simulink model "MRG1x_17B_ERP_030_00_Star23_xx_M256xx_910_x64_RB_Test"  (Simulink 7.8)
settings: Solver=ode45  SolverMode=SingleTasking  StartTime=0.0  StopTime=10.0  RelTol=1e-3
PreLoadFcn:
  | MRG1x_17B_ERP_030_00_Star23_xx_M256xx_910_x64_InitFcn
undefined symbols (not defined in the file or in its folder): ECM
(part 2 of 2)

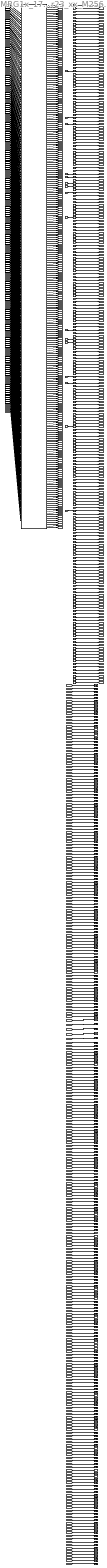
== system MRG1x_17B_ERP_030_00_Star23_xx_M256xx_910_x64_RB_Test/MRG1x_17B_ERP_030_00_Star23_xx_M256xx_910_x64_wrapper ==
  AAP : Inport
  AC_HtrVlv_Front_Req : Inport  Port=2
  AGC_ASSStop_Mode : Inport  Port=3
  AGC_DTREngCutOff_Mode : Inport  Port=4
  AGKInit_Mode : Inport  Port=5
  APP : Inport  Port=6
  AT2_Mode : Inport  Port=7
  AdapAltitudeTempCorr_Coef : Inport  Port=8
  AirFilOutTp_Tp : Inport  Port=9
  AmbAirP_P : Inport  Port=10
  AmbAirTp_Tp : Inport  Port=11
  Bat_Volt : Inport  Port=12
  CacInTp_Tp : Inport  Port=13
  DFI_OprState : Inport  Port=14
  DFSO_Mode : Inport  Port=15
  Dspl_EngShutOff_Time : Inport  Port=16
  ECT : Inport  Port=17
  ECTOut : Inport  Port=18
  ECU_Temp : Inport  Port=19
  EM2_Cool_Req : Inport  Port=20
  EM2_InvrtTemp : Inport  Port=21
  Ecu_St : Inport  Port=22
  Emmo_VoltLinkPN48 : Inport  Port=23
  EngClpmp_FlgOnReq : Inport  Port=24
  EngClpmp_PercPwrReq : Inport  Port=25
  EngCoolTp_Tp : Inport  Port=26
  EngCoolTp_TpMdl : Inport  Port=27
  EngOilP_P : Inport  Port=28
  EngOilTp_Tp : Inport  Port=29
  EngShutOff_Time : Inport  Port=30
  Eng_Actl_OpMode : Inport  Port=31
  Eng_Cyc_Time : Inport  Port=32
  Eng_Fuel_Mass_Flow_Calc : Inport  Port=33
  Eng_RelLoad : Inport  Port=34
  Eng_RelLoad_Req : Inport  Port=35
  Eng_Run_Mode : Inport  Port=36
  Eng_Spd : Inport  Port=37
  Eng_State_Actl : Inport  Port=38
  Eng_Trq : Inport  Port=39
  Eng_Trq_Ind : Inport  Port=40
  Err_ECT_low : Inport  Port=41
  Exh_Temp : Inport  Port=42
  ExtAir_Temp_Raw : Inport  Port=43
  FRT_Sens : Inport  Port=44
  FirstStrt_Mode_EE : Inport  Port=45
  Fu_Mp1 : Inport  Port=46
  Fuel_Temp : Inport  Port=47
  Gear_State : Inport  Port=48
  HDC_HybAggr_State : Inport  Port=49
  Hepm_PwrMax48VEcm : Inport  Port=50
  Hvac_StDefrstAcv : Inport  Port=51
  IC_Knk_Red_Avg : Inport  Port=52
  IC_Knk_Red_Avg_Actv : Inport  Port=53
  IMAT : Inport  Port=54
  Idle_Mode_Req : Inport  Port=55
  IgnSwRun_Mode : Inport  Port=56
  IgnSwStrtr_Mode : Inport  Port=57
  Ign_Mode : Inport  Port=58
  Injr_Tp : Inport  Port=59
  IntkAir_Temp : Inport  Port=60
  K15 : Inport  Port=61
  LIN_CF_Spd_Req : Inport  Port=62
  LIN_CP_ECP4TransActlSpd : Inport  Port=63
  LIN_CP_ECP4TransVoltStat : Inport  Port=64
  MAF : Inport  Port=65
  Net_EBoost_CurrCons : Inport  Port=66
  Odo_Abs_Long : Inport  Port=67
  Pnct48V_VoltMinThdShutDwnEcm : Inport  Port=68
  ScrcmDos_THeatrPmpAftRunReq : Inport  Port=69
  Shuttr_Pos_Req_I : Inport  Port=70
  TCM_Oil_Temp : Inport  Port=71
  TM_ShttrDeIcing_ECTRef_I : Inport  Port=72
  TM_Shttr_TjaErrIrrv_LIN : Inport  Port=73
  TmClpmp_LtCcrGbRsgTpQvolReq : Inport  Port=74
  TmFan_MalfFlg : Inport  Port=75
  TmHiTp_ThOpenSts : Inport  Port=76
  Tm_FlgEngOilHiPReq : Inport  Port=77
  Trans_OilTempHigh_Mode : Inport  Port=78
  TrbInTp_Tp : Inport  Port=79
  TrqSetIgn_Mode_Req : Inport  Port=80
  TrqSetRes_Mode_Req : Inport  Port=81
  VehMass_Wght_Pred : Inport  Port=82
  Veh_Spd : Inport  Port=83
  ag_CamsftExhSp : Inport  Port=84
  ag_CamsftIntkSp : Inport  Port=85
  flg_ChrgrAirCcrAcv : Inport  Port=86
  flg_PAFGCoolFanLinMod : Inport  Port=87
  n_Eng : Inport  Port=88
  perc_PAFGCoolFanLinReq : Inport  Port=89
  tp_ExhAtExhMnfld : Inport  Port=90
  Dlay_ECTOut : UnitDelay  SampleTime=-1
  Dlay_EngShutOff_Time : UnitDelay  SampleTime=-1
  Dlay_Exh_Temp : UnitDelay  SampleTime=-1
  Dlay_FirstStrt_Mode_EE : UnitDelay  SampleTime=-1
  Dlay_IgnSwRun_Mode : UnitDelay  SampleTime=-1
  Dlay_LIN_CF_Spd_Req : UnitDelay  SampleTime=-1
  Dlay_Shuttr_Pos_Req_I : UnitDelay  SampleTime=-1
  Dlay_TM_ShttrDeIcing_ECTRef_I : UnitDelay  SampleTime=-1
  Dlay_TM_Shttr_TjaErrIrrv_LIN : UnitDelay  SampleTime=-1
  Dlay_TmClpmp_LtCcrGbRsgTpQvolReq : UnitDelay  SampleTime=-1
  Dlay_TmFan_MalfFlg : UnitDelay  SampleTime=-1
  Dlay_TmHiTp_ThOpenSts : UnitDelay  SampleTime=-1
  Dlay_Tm_FlgEngOilHiPReq : UnitDelay  SampleTime=-1
  Dlay_flg_ChrgrAirCcrAcv : UnitDelay  SampleTime=-1
  Dlay_flg_PAFGCoolFanLinMod : UnitDelay  SampleTime=-1
  Dlay_perc_PAFGCoolFanLinReq : UnitDelay  SampleTime=-1
  const_ACCompr_RunMode_Plaus : Constant  Value=0
  const_AC_HtrVlv_Front_ReqSq : Constant  Value=0
  const_AirFilOutTp_Sq : Constant  Value=0
  const_AmbAirP_Sq : Constant  Value=0
  const_AmbAirTp_Sq : Constant  Value=0
  const_Bms48_StCntctrD : Constant  Value=0
  const_CacInTp_Sq : Constant  Value=0
  const_CarHtr_EngStrt_Mode : Constant  Value=0
  const_Com_HPP_DrvProg : Constant  Value=0
  const_Crash_Mode : Constant  Value=0
  const_DTM_Mode : Constant  Value=0
  const_Diag_DsblCntr_Resp : Constant  Value=0
  const_DiagcTstr_EngClpmpActFlg : Constant  Value=0
  const_DiagcTstr_EngClpmpReqPwm : Constant  Value=0
  const_DiagcTstr_PcdOilPDeacvnKmFlg : Constant  Value=0
  const_DrProgram : Constant
  const_ECF_Pwr_Req : Constant  Value=0
  const_EM2_Cool_ReqSq : Constant  Value=0
  const_EM2_InvrtTempSq : Constant  Value=250
  const_EOM_Actl_OpMode : Constant  Value=0
  const_Emmo_PwrRecupForEbstrAvl : Constant  Value=0
  const_Emmo_PwrRecupForEbstrAvlSq : Constant  Value=0
  const_Emmo_VoltLinkPN48Sq : Constant  Value=0
  const_EngClpmp_FlgOnReqSq : Constant  Value=0
  const_EngClpmp_PercPwrReqSq : Constant  Value=0
  const_EngCoolThOutTp_Tp : Constant  Value=0
  const_EngCoolTp_Sq : Constant  Value=0
  const_EngHood_Plaus_Mode : Constant  Value=0
  const_EngOilP_Sq : Constant  Value=0
  const_EngOilTp_Sq : Constant  Value=0
  const_ErrErs_Mode : Constant  Value=0
  const_Err_ECU_Temp_Mode : Constant  Value=0
  const_Err_EngShutOff_Time : Constant  Value=0
  const_Err_MAF_Mode : Constant  Value=0
  const_Exh_Temp_Err_Mode : Constant
  const_FirstStrt_Mode : Constant  Value=0
  const_Hepm_PwrMax48VEcmSq : Constant  Value=0
  const_Hpmc_StPlgnOpmdReq : Constant  Value=0
  const_Hvac_StDefrstAcvSq : Constant  Value=0
  const_LIN_CP_ECP4StEltlErr : Constant  Value=3
  const_LIN_CP_ECP4TransActlSpdSq : Constant  Value=0
  const_LIN_CP_ECP4TransBlkErr_State : Constant  Value=0
  const_LIN_CP_ECP4TransCurr : Constant  Value=0
  const_LIN_CP_ECP4TransCurrSq : Constant  Value=0
  const_LIN_CP_ECP4TransDryRunErr_State : Constant  Value=0
  const_LIN_CP_ECP4TransMon_StateSq : Constant  Value=0
  const_LIN_CP_ECP4TransOvrCurrErr_St : Constant  Value=0
  const_LIN_CP_ECP4TransOvrTpErr_State : Constant  Value=0
  const_LIN_CP_ECP4TransPostRun_StateSq : Constant  Value=0
  const_LIN_CP_ECP4TransPwmIn_StateSq : Constant  Value=0
  const_LIN_CP_ECP4TransRpmRedStat : Constant
  const_LIN_CP_ECP4TransTgtSpdSq : Constant  Value=0
  const_LIN_CP_ECP4TransTpSq : Constant  Value=0
  const_LIN_CP_ECP4TransVoltErr_State : Constant  Value=0
  const_LIN_CP_ECP4TransVoltStatSq : Constant  Value=0
  const_Net_EBoost_CurrConsSq : Constant  Value=0
  const_Pn14Bat_Typ : Constant
  const_Pnct48V_VoltMinThdShutDwnEcmSq : Constant  Value=0
  const_Prcs_DiagRstFlg : Constant  Value=0
  const_RotVlvMalf_Mode : Constant  Value=0
  const_TCM_Oil_TempSq : Constant  Value=0
  const_TM_RegenActive_Mode : Constant  Value=0
  const_TM_Shttr_TjaErrIrrv_LINSq : Constant  Value=0
  const_ThrInTp_Sq : Constant  Value=0
  const_TmClpmp_LtCcrGbRsgTpQvolReqSq : Constant  Value=0
  const_TmClpmp_ThDiagClpmpPWM : Constant  Value=0
  const_TmFan_MalfFlgSq : Constant  Value=0
  const_TmMdl_TpTchQhtCor : Constant  Value=0
  const_TmPredCtl_EcTpSp : Constant  Value=0
  const_TmTh_AcvThDiagOpgFlg : Constant  Value=0
  const_Trlr_State : Constant  Value=0
  const_Trlr_StateSq : Constant  Value=0
  const_Veh_Spd_Err_Mode : Constant  Value=0
  const_WiprOutOfParkPosn : Constant  Value=0
  const_flg_PremAirGrdtFai : Constant  Value=0
  const_flg_PremAirPosFrameAcv : Constant  Value=0
  const_flg_PremAirTmDirt : Constant  Value=0
  const_flg_PremAirTmDirtT : Constant  Value=0
  const_flg_PremAirTmOpen : Constant  Value=0
  const_flg_TestDiagTmLtCcrVlvIcoMod : Constant  Value=0
  const_flg_TestDiagTmLtCcrVlvIcoReq : Constant  Value=0
  const_flg_TmHwCptSwtlEnag : Constant  Value=0
  const_modIn_Trigger_Cyl_Cntr : Constant  Value=0
  const_timePostdrive : Constant  Value=0
  eeprom_TM_CCRGAEATHi : Constant  Value=0
  eeprom_TM_CCRGAEATLo : Constant  Value=0
  eeprom_TM_CCRGAEATMid : Constant  Value=0
  eeprom_TM_CCRGA_Hi : Constant  Value=0
  eeprom_TM_CCRGA_Lo : Constant  Value=0
  eeprom_TM_CCRGA_Mid : Constant  Value=0
  eeprom_TM_CCRGA_act : Constant  Value=0
  eeprom_TM_ECT_Ref_Cntr_HT : Constant  Value=0
  eeprom_TM_ECT_Ref_Cntr_LT : Constant  Value=0
  eeprom_TM_LTCoolPump_RunTime6 : Constant  Value=0
  eeprom_TOil_ShutOff : Constant  Value=0
  eeprom_TmEcTpSp_CtrEcuTp{0..9} (10 alike) : Constant  Value=0
  eeprom_TmEcTpSp_TpEcuCtrDiRam : Constant  Value=0
  eeprom_TmHi_FacTCor2Ee : Constant  Value=0
  eeprom_TmPcdLrng_CtlrFctCoefY100 : Constant  Value=0
  eeprom_TmPcdLrng_CtlrFctCoefY20 : Constant  Value=0
  eeprom_TmPcd_EepromPDeacvnOdoS : Constant  Value=0
  eeprom_TmPmp_TpQhtTchDram : Constant  Value=0
  sfunction : S-Function  FunctionName=MRG1x_17B_ERP_030_00_Star23_xx_M256xx_910_x64  Parameters=AV_AgkSp10ms_EngSpdActive_P,AV_AgkSpSeg_EngSpdActive_P,FW_TM_AC_RVPWR,TmSigIf_AmbAirTpSqThd_P,TmSigIf_ChrgrAirCcrAcvFlg_P,TmSigIf_EctErrSq_P,TmSigIf_EctIniSq_P,TmSigIf_EnaFlgStopDiMod_P,TmSigIf_OilPmpPWMThd_P,TmSigIf_OilTpSqValHi_P,TmSigIf_OilTpSqValLo_P,TmSigIf_StPrioReq12_P,TmSigIf_StrtrDlyT_P,TmSigIf_StWpReq12_P,TmSigIf_TpCmprOutMdl2Sq_P,Tm_CpcCodMdlActnCoef_P,Tm_ExhTpSelctr_P,Tm_LtCcrCacTpSwtFlg_P,Tm_ProdModEngNThd_P,Tm_CpcErrEltFanDlyT_P,Tm_CpcErrEltShttrDlyT_P,Tm_ErrEntryEltCompAct_P,TmFan_CpcErrPahLinFanEna_P,TmFan_StEcuCpcActrErrPahEna_P,TmShttr_CpcErrPahLinShttrEna_P,TmClpmp_BlkErrEnaFlg_P,TmClpmp_BlkErrSt_P,TmClpmp_DryRunErrEnaFlg_P,TmClpmp_DryRunErrSt_P,TmClpmp_Ecp4ComErrMsgLostDeb_P,TmClpmp_Ecp4MsgLostSq_P,TmClpmp_EltErrSt_P,TmClpmp_EltlErrEnaFlg_P,TmClpmp_ErrDebT_P,TmClpmp_ErrIrrvDlyT_P,TmClpmp_ErrMaskIrrv_P,TmClpmp_ErrMaskRvsb_P,TmClpmp_ErrRvsbDlyT_P,TmClpmp_ErrSetAcvFlg_P,TmClpmp_MaskEcp4MsgLostSq_P,TmClpmp_OverCurErrEnaFlg_P,TmClpmp_OverCurErrSt_P,TmClpmp_OverTpErrSt_P,TmClpmp_RefErrEna_P,TmClpmp_RpmRedStEnaFlg_P,TmClpmp_SqLoVal_P,TmClpmp_SqMax_P,TmClpmp_SqMin_P,TmClpmp_StEltlErr_P,TmClpmp_TDebElClpmpBlkErr_P,TmClpmp_TDebElClpmpDryRunErr_P,TmClpmp_TDebElClpmpEltlErr_P,TmClpmp_TDebElClpmpOverCurErr_P,TmClpmp_TDebElClpmpVoltErr_P,TmClpmp_VoltErrEnaFlg_P,TmClpmp_VoltErrErrSt_P,TmPmp_ClpmpBatVActErrThd_P,TmPmp_ClpmpErrDebT_P,TmPmp_ClpmpHiNErrThr1_P,TmPmp_ClpmpHiSpdErrAcvFlg_P,TmPmp_ClpmpLoNErrThr1_P,TmPmp_ClpmpLoSpdErrAcvFlg_P,TmPmp_ClpmpNActErrThd_P,TmPmp_ClpmpPn48VActErrThd_P,TmPmp_EngClpmpLinReqPwmLim_P,TmPmp_TDebErrEnaNErrLinReqPwm_P,TmClpmp_AcvFlgEngClpmp_P,fac_TmDrvpRampOfsTpCooltFanLo_P,fac_TmTpAmbOfsTpCooltFanLo_A,fac_TmTpAmbOfsTpCooltFanLo_L,fac_TmVPwrOfsFanLo_A,fac_TmVPwrOfsFanLo_L,fac_TmVTpEcuFan_A,fac_TmVTpEcuFan_L,FanDynRideEna_P,flg_MesCameoInca_P,flg_TmRelsTpCooltHtDplFanLo_P,FW_TM_CAF_CT_AC_Max,FW_TM_CAF_CT_DPF_RegenWCR_Req,FW_TM_CAF_CT_DPFPrevReq_T,FW_TM_CAF_CT_DPFReg_SelC,FW_TM_CAF_CT_ECTIncTrlr,FW_TM_CAF_CT_ECTModLEngSpd,FW_TM_CAF_CT_ECTModLGradt_En,FW_TM_CAF_CT_ECTModLGradtDelta,FW_TM_CAF_CT_ECTModLGradtDeltaT,FW_TM_CAF_CT_ECTModLGradtDly,FW_TM_CAF_CT_ECTModLGradtOfs,FW_TM_CAF_CT_Eng_RelLoad,FW_TM_CAF_CT_EngComp_Max,FW_TM_CAF_CT_Exh_Temp_T,FW_TM_CAF_CT_ExtAir_Temp,FW_TM_CAF_CT_FanLoadInc_Req,FW_TM_CAF_CT_GenrHiFanHi,FW_TM_CAF_CT_GenrHiFanLo,FW_TM_CAF_CT_GenrHiVoltGrdtMax,FW_TM_CAF_CT_GenrHiVoltGrdtStrt,FW_TM_CAF_CT_IntkAir_Temp,FW_TM_CAF_CT_NT_Max,FW_TM_CAF_CT_Pwr_TFilT,FW_TM_CAF_CT_RoModeReq,FW_TM_CAF_CT_TGET_Max,FW_TM_CAF_CT_VS,FW_TM_CAF_DPF_ACCntl_dis,FW_TM_CAF_ECT2Lim,FW_TM_CAF_ECTDelayT2,FW_TM_CAF_ECTFilT,FW_TM_CAF_ECTLim,FW_TM_CAF_ECTLim_sstL2,FW_TM_CAF_ECTMod_Config,FW_TM_CAF_Hyst_En,FW_TM_CAF_HystLimFilt,FW_TM_CAF_HystTFilt,FW_TM_CAF_HystVSpdH,FW_TM_CAF_HystVSpdL,FW_TM_Coolfan2_Enable,FW_TM_CoolHybr_EMxiTemp_LowpTim,FW_TM_CoolHybr_enable,FW_TM_CoolHybr_Err_Mode_Delay,FW_TM_ECF_DPFPwrReq_enable,FW_TM_ECF_DPFPwrReq_FirESpd_T,FW_TM_ECF_DPFPwrReqMan_Val,FW_TM_ECTReq_DelayTime,FW_TM_ECTSetp_Mode,idx_TmSelVehVarOfsFanLoEna_P,idx_TmSelVehVarTpEcuFanSel_P,KF_TM_CAF_EngPwrInd_22,KF_TM_CAF_PwrInd_VS33,KF_TM_ECF_DPFPwrReq_FirESpd,KL_TM_CAF_CT_DPFMaxReqVSpd,KL_TM_CAF_CT_DPFPrevReq_EAT,KL_TM_CAF_CT_DPFPrevReq_ECT,KL_TM_CAF_CT_ECT_H_08B,KL_TM_CAF_CT_ECT_HOffs_08B,KL_TM_CAF_CT_ECT_L_08B,KL_TM_CAF_CT_ECT_L_L2_08B,KL_TM_CAF_CT_ECTShift,KL_TM_CAF_CT_Fuel_Temp_08B,KL_TM_CAF_CT_SenOil_Temp_Req,KL_TM_CAF_CT_VSDly04,KL_TM_CAF_ECU_Temp_06,KL_TM_CAF_IntkAir_Temp_04,KL_TM_ECTTime_04,KL_TM_EMx_InvrtTemp_04,req_TmTpCooltHtStopMaxFan_A,req_TmTpCooltHtStopMaxFan_L,req_TmTpScrRegrEngStopMaxFan_P,req_TmTpScrRegrToFan_A,req_TmTpScrRegrToFan_L,sst_TM_CAF_CT_EAT,sst_TM_CAF_CT_ECT_H,sst_TM_CAF_CT_ECT_HOffs,sst_TM_CAF_CT_ECT_L,sst_TM_CAF_CT_ECT_L_L2,sst_TM_CAF_CT_ECTOut,sst_TM_CAF_CT_EngSpd,sst_TM_CAF_CT_FIRate_DPFPwr,sst_TM_CAF_CT_Fuel_Temp,sst_TM_CAF_CT_PwrInd03,sst_TM_CAF_CT_SenOilTemp,sst_TM_CAF_CT_VS03,sst_TM_CAF_CT_VS04,sst_TM_CAF_CT_VSpd_DPFMax,sst_TM_CAF_CT_VSpd_ECTShi,sst_TM_CAF_ECU_Temp6,sst_TM_CAF_ECU_Temp6_BR,sst_TM_CAF_IntkAir_Temp4,sst_TM_ECTTime,sst_TM_EMx_InvrtTemp_04,sst_TM_EngSpd_02,sst_TM_EngTrqInd_02,t_TmDrvpRelsFanLoAcvtDly_P,t_TmDrvpRelsFanLoDeacvtDly_P,t_TmEngPwrGrdtFallFanLoFil_P,t_TmEngPwrGrdtRisngFanLoFil_P,t_TmTpAirAspFanFild_P,t_TmTpAirAspFanFildAcvt_P,Tm_CafDynRideAccrGradtDlyT_P,Tm_CafDynRideOfsAccrGrdtThd_A,Tm_CafDynRideOfsAccrGrdtThd_L,Tm_CafDynRideOfsAccrThd_A,Tm_CafDynRideOfsAccrThd_L,Tm_CafDynRideOfsDlyT_P,Tm_CafDynRideOfsTp_P,Tm_CtrDpfRgnFanPwrReqInct_L,Tm_CtrDpfRgnFanPwrReqInct_P,Tm_CtrDpfRgnFanPwrReqInctX_A,Tm_CtrDpfRgnFanPwrReqMaxLim_P,Tm_FacDpfRgnFanPwrReqCorrn_L,Tm_FacDpfRgnFanPwrReqCorrnX_A,Tm_FacDpfRgnFanPwrReqInct_P,Tm_FacDynRideOfsTpCooltFanLo_A,Tm_FacDynRideOfsTpCooltFanLo_L,Tm_FanGpfRgnSrvVMax_P,Tm_FanGpfRgnTpSeln_P,Tm_FanGpfRstTDly_L,Tm_FanGpfRstTDlyX_A,Tm_IdleRelsTOffDly_P,Tm_IdleRelsTOnDly_P,Tm_IdleRelsVehV_P,Tm_PwrDpfRgnIntegdFanReq_L,Tm_PwrDpfRgnIntegdFanReqX_A,Tm_PwrGpfRgnIntegdFanReq_M,Tm_PwrGpfRgnIntegdFanReqX_A,Tm_PwrGpfRgnIntegdFanReqY_A,Tm_PwrRgnIntegdFanSeln_P,TmEngPwrOfsTpCooltFanLoFilThd_P,TmFan_BatTyp_P,TmFan_BrkAMSCycDlyT_P,TmFan_BrkAMSCycDlyTRunOn_P,TmFan_BrkAMSCycHiLoNSp_P,TmFan_BrkAMSCycHiValN_P,TmFan_BrkAMSCycLoNSp_P,TmFan_BrkAMSCycOfsTp_P,TmFan_CtrCodModVehM0Lrg_P,TmFan_CtrCodModVehM0Mean_P,TmFan_CtrCodModVehM0Mild_P,TmFan_CtrCooltReqHiThd_P,TmFan_CtrCooltReqLoThd_P,TmFan_CtrExhTpFanReq_M,TmFan_CtrGbOilTpFanReq1_L,TmFan_CtrHeatIntglFanReq_L,TmFan_CtrHeatIntglFanReqX_A,TmFan_CtrQhtTchTpFanReq_L,TmFan_DPFPwrReq_A,TmFan_DPFPwrReq_L,TmFan_Em2InvTpSqLoThd_P,TmFan_FacAmbAirTpDpfRgnLoaFan_A,TmFan_FacAmbAirTpDpfRgnLoaFan_L,TmFan_FacCoolgFanStrtCor_P,TmFan_FacExtAirTp_A,TmFan_FacExtAirTp_L,TmFan_FacHeatIntglFanReq_M,TmFan_FacHeatIntglFanReqX_A,TmFan_FacHeatIntglFanReqY_A,TmFan_FlgSmkPrevnManEna_P,TmFan_GbTpFlgAcv_P,TmFan_HdcStErrEna_P,TmFan_HdcStSelnFanAcvn_P,TmFan_HybCptReqFlgAcv_P,TmFan_MAF_P,TmFan_MaxSeln3SDi_P,TmFan_MaxVoltBatTyp1_P,TmFan_MaxVoltBatTyp2_P,TmFan_MCodModVehM0_P,TmFan_MVehPLoaMFanReqDpl_A,TmFan_PAvgPResvCoolgFanReqFil_A,TmFan_PercIntEngFanReq_A,TmFan_PwmEctIdleHi08Bit_M,TmFan_PwmEctIdleLo08Bit2_M,TmFan_PwmEctIdleLo08Bit_M,TmFan_QInjSelFan1_P,TmFan_RateIntEngFanReq_L,TmFan_SpMaskHiPP_P,TmFan_StDpfPwrReqFan1_P,TmFan_StDrvProg_P,TmFan_StEcu_P,TmFan_TAvgPResvCoolgFanReqFil_L,TmFan_TDlyCooltReqOff_P,TmFan_TDlyCooltReqOn_P,TmFan_TEctHiFilFall_P,TmFan_TEctHiFilRise_P,TmFan_TEctLoFilFall2_P,TmFan_TEctLoFilFall_P,TmFan_TEctLoFilRise2_P,TmFan_TEctLoFilRise_P,TmFan_TExhTpFilFall_P,TmFan_TExhTpFilRise_P,TmFan_THiLoaTp_P,TmFan_TMAF_P,TmFan_TpAirIntk_P,TmFan_TpExhFanReqX_A,TmFan_TpExhFanReqY_A,TmFan_TpExhTpHysFall_P,TmFan_TpExhTpHysRise_P,TmFan_TpGbOilFanReq1_A,TmFan_TpQhtTchFanReq_A,TmFan_TpQhtTchSeln_P,TmFan_TpVehPLoaMFanReqDpl_L,TmFan_TVehVResvCoolgFanReqFil_L,TmFan_TVLimVehMPredValDly_P,TmFan_VehNOfPwmEctHiY_A,TmFan_VehNOfPwmEctLoY_A,TmFan_VVehLimVehMPredVal_P,TmFan_VVehVResvCoolgFanReqFil_A,TmFanIdleRels_FlgMod_P,TmFanIdleRels_VehNMaxThd_P,TmFanIdleRels_VehNMinThd_P,TmFanSmkPrevn_NReqTDly_P,TmFanSmkPrevn_PmpAcvdTDly_P,TmFanSmkPrevn_VehNMaxThd_P,TmFanSmkPrevn_VehNMinThd_P,TmPredCtl_FanNReq_M,TmPredCtl_FanNReqFac_A,TmPredCtl_FanNReqFac_L,TmPredCtl_FanNReqFallFilT_P,TmPredCtl_FanNReqMaskEnaSt1_P,TmPredCtl_FanNReqRisngFilT_P,TmPredCtl_FanNReqXdir_A,TmPredCtl_FanNReqYdir_A,TmSmkFmtPrevn_FanNReq_P,TmSmkPrevn_StSelnManEna_P,TmSmkPrevn_WiprPosnEveCtr_P,TmSmkPrevn_WiprPosnTDly_P,tp_TmAmbOfsTpCooltLoFanLo_A,tp_TmAmbOfsTpCooltLoFanLo_L,tp_TmDrvpMaxOfsTpCooltFanLo_P,tp_TmEngPwrOfsTpCooltFanLo16_A,tp_TmEngPwrOfsTpCooltFanLo16_L,FW_DTM_Mode_En,FW_GearStateControl_DMx,FW_GearStateControl_RMn,FW_SG_enable,FW_TM_ASSStopMode_OffDly,FW_TM_CAF_AppLoLim,FW_TM_CAF_ASSStopDelay_dis,FW_TM_CAF_CoolFanReqNT_en,FW_TM_CAF_CoolFanVeloChar,FW_TM_CAF_CV_DTM_ETC_UpLim,FW_TM_CAF_CV_ErrEnable,FW_TM_CAF_EHoodCntl_en,FW_TM_CAF_EngRunDelay_dis,FW_TM_CAF_EngRunDelay_en,FW_TM_CAF_GearPwrTransDelay,FW_TM_CAF_HDC_EDrive,FW_TM_CAF_HDC_EDrive_en,FW_TM_CAF_IgnSwRunMode_dis,FW_TM_CAF_PwrFree_Cntl,FW_TM_CAF_UBatMin,FW_TM_CAF_VL_elViscoFan_en,FW_TM_CAF_VSpdLimDelay_en,FW_TM_CAF_VSpdLimH,FW_TM_CAF_VSpdLimL,FW_TM_CAF_VSpdLoLim,FW_TM_CoolFan_DTC,FW_TM_CoolFan_DTM,FW_TM_CoolFan_DTM_0,FW_TM_CoolFan_DTM_Pos,FW_TM_CoolFan_Eng_Run_Mode_T,FW_TM_CoolFan_ErrPos,FW_TM_CoolFan_Ramp_en,FW_TM_CoolFan_Req_Min,FW_TM_ECTOut_Max,FW_TM_EcuTempErr_en,FW_TM_OilTemp_Switch,FW_TM_Sens_Oil_Temp_Max,FW_TM_Shuttr_Pos_Req_LowLim,KL_CoolFanPwrReq_Lim,KL_TM_Luefter7_S16,sst_CoolFanPwrReq_Lim,sst_TM_CAF_VehSpd_Lu7,sst_TM_CoolFan_MAF_Req,TmFan_FlgCrashMdlEnaFanReqCtl_P,TmFan_FlgLinFanErrDispFbEna_P,TmFan_FlgReqManSel_P,TmFan_PercFanReqDisLimnVPwr_P,TmFan_PercFanReqEnaLimnVPwr_P,TmFan_PercFanReqLimnVPwr_M,TmFan_PwrFanReqLimn_A,TmFan_TLinFanErrDispFbReqDly_P,TmFan_TPercFanReq1_P,TmFan_TPercFanReq2_P,TmFan_TPercFanReq3_P,TmFan_TPercFanReq4_P,TmFan_VFanReqLimn_A,TmFanLin_ClfanPwrReqLim_A,TmFanLin_ClfanPwrReqLim_L,Tm_FuEngRPM_A,Tm_FuEngTp_A,Tm_FuMp1_A,Tm_FuMpEngRpmOfs1_M,Tm_FuMpEngTpFac1_M,Tm_FuMpTpInInjr1_M,Tm_FuTpDifMax_P,Tm_FuTpDifMin_P,Tm_FuTpInInjr_A,Tm_FuTpSwt_P,TmClpmp_AcvThDiagAcvnFlg_P,TmClpmp_EngNMin_P,TmClpmp_FlgAcvtDefrstAcv_P,TmClpmp_PmpCtlAmbAirEctTpFacX_A,TmClpmp_PmpCtlAmbAirEctTpFacY_A,TmClpmp_PmpCtlAmbAirEctTpFac_M,TmClpmp_PmpCtlEngNBpr_A,TmClpmp_PmpCtlEngNTrqPwm_M,TmClpmp_PmpCtlEngTrqBpr_A,TmClpmp_PmpCtlGbTpQvolBpr_A,TmClpmp_PmpCtlGbTpQvolPwm_L,TmClpmp_PmpCtlGbTpQvolSqMax_P,TmClpmp_PmpCtlGbTpQvolSqMin_P,TmClpmp_PmpCtlHvacAcvFlg_P,TmClpmp_PmpCtlHvacPwmSqMax_P,TmClpmp_PmpCtlHvacPwmSqMin_P,TmClpmp_PmpCtlHvacPwm_P,TmClpmp_PmpCtlPercPwrEctAmbAirTpFacX_A,TmClpmp_PmpCtlPercPwrEctAmbAirTpFacY_A,TmClpmp_PmpCtlPercPwrEctAmbAirTpFac_M,TmClpmp_PmpCtlPercPwrReqBpr_A,TmClpmp_PmpCtlPercPwrReqPwmMax_P,TmClpmp_PmpCtlPercPwrReqPwm_L,TmClpmp_PmpCtlPrtclFilRgnAftRunTDly_P,TmClpmp_PmpCtlPrtclFilRgnCorrnPercX_A,TmClpmp_PmpCtlPrtclFilRgnCorrnPerc_L,TmClpmp_PmpCtlPrtclFilRgnTchPercX_A,TmClpmp_PmpCtlPrtclFilRgnTchPerc_L,TmClpmp_PmpCtlTCorrdPwmX_A,TmClpmp_PmpCtlTCorrdPwm_L,TmClpmp_ThAdpnReqPwm_P,TmClpmp_VehNMax_P,TmPmp_AatWhtngFac_A,TmPmp_AatWhtngFac_L,TmPmp_BprHiEcTp_A,TmPmp_BprLoEcTp_A,TmPmp_CtlReqHiEcTpPerc_L,TmPmp_CtlReqLoEcTpPerc_L,TmPmp_EngCooltTpMax_P,EngOvrheatdProtn_DynRideLoa_P,EngWtr_TpVrntOfs_P,FW_Cod_Func_BoilProt_en,FWDLYKOCH,FWMAFRL,FWMLKOCHMN,FWOILSNAENA,FWTLKOCHMX,FWTMOTKOCH,FWTOELKOCH,FWTPKOCH,KLFKOCH,KLFKOCH2,KLMXKOCH,Mask_ExtdRelLoadOvrHtgPrvn_P,n_RelLoadOvrHtgPrvn2_L,n_RelLoadOvrHtgPrvn3_L,n_RelLoadOvrHtgPrvn_L,OvrheatgFacVehV_L,OvrheatgVehV_A,SnsrOil_TpVrntOfs_P,sst_ECTOut,sst_SenOilTemp2,t_RelLoadOvrHtgPrvnCorrn_P,Tm_ClpmpErrMask_P,Tm_EngClpmp4ActNSqThd_P,Tm_EngClpmp4MsgLostSq_P,Tm_EngClpmp4NThdRed_P,Tm_EngClpmp4TranDryRunErrSt_P,Tm_EngClpmp4VoltSqThd_P,Tm_EngClpmp4VoltThdRed_P,Tm_EngCoolThOutTp_L,Tm_EngCoolThOutTpMax_P,Tm_EngCoolThOutTpMin_P,Tm_EngCoolThOutTpX_A,Tm_RelLoaCoolgPrevn_L,Tm_RelLoaCoolgPrevnX_A,Tm_RelLoaEnaDlyTClpmpMalf_A,Tm_RelLoaEnaDlyTClpmpMalf_L,Tm_RelLoaEngClpmpDryRunErr_L,Tm_RelLoaEngClpmpMalf_L,Tm_RelLoaTpFacClpmpMalf_A,Tm_RelLoaTpFacClpmpMalf_L,tp_EngWtr_A,tp_RelLoadOvrHtgPrvn2_A,tp_RelLoadOvrHtgPrvn_A,tp_RelLoadOvrHtgPrvn_L,tp_RelLoadOvrHtgPrvn_M,NISTV08,VCANV16,FW_TMManKE,FW_TMManKE_en,FW_TMSelDFI,FW_TM_EAT_CTLim,FW_TM_ECT_AirTempPREV_sel,FW_TM_ECT_CTLim,FW_TM_ECT_LoadOilSel_Hi,FW_TM_ECT_LoadOilSel_Lo,FW_TM_ECT_Ref_DE,FW_TM_ECT_Ref_LoadOil_Hi,FW_TM_ECT_Ref_Mode,FW_TM_ECT_Ref_Prev_Hi,FW_TM_ECT_Ref_Prev_Lo,FW_TM_ECT_Ref_VSLoadReset,FW_TM_Ref_FIRate_Mode,FW_TM_Ref_Load_Mode,FW_TM_Ref_Prev_MAF,FW_TM_ST_ECT_CTLim,FW_TM_T_Ref_Prev_Hi,FW_TM_T_Ref_Prev_HiFast,FW_TM_T_Ref_Prev_Hi_Dly,FW_TM_T_Ref_Prev_Lo_Dly,sst_TM_LOAD_PREV,TmDmd_QInjSelMinLoa_P,TmDmd_SelIntkAirTp_P,TmDmd_StEcuMinLoa_P,TmDmd_TFilLoaFallTpCorOff_P,TmDmd_TFilLoaFallTpCorOn_P,TmDmd_TFilLoaRiseTpCorOff_P,TmDmd_TFilLoaRiseTpCorOn_P,TmDmd_TpCorHysHi_P,TmDmd_TpCorHysLo_P,TmDmd_TRefPrevLoNBpr_A,TmDmd_TRefPrevLoNTq_M,TmDmd_TRefPrevLoTqBpr_A,TmTmCntlAcvnDlyT_P,TmTpTmCntlAcvnThd_P,TM_AirTemp_FacPREV_sst_04,TM_AirTemp_FAC_PREV_KL,TM_ECT_Ref_PREV_KF78_S8,TM_NIST_PREV_07,TM_VS_FAC_04,TM_VS_FAC_PREV_KL,FW_TM_ECT_Ref_Mech,FW_TM_ECT_Ref_Disable,FW_TM_ECT_Ref_DisableDPF,FW_TM_ECT_Ref_StatistT,FW_TM_ECTDis_H,FW_TM_ECTDis_L,FW_TM_ECTDis_L_DPF,FW_TM_ECTDisIVal,FW_TM_ECTEnIVal,FW_TM_Ref_Err_en,FW_TMManECTCod,FW_TMManECTRef,TM_EATDis_H_DPF04,TM_ECTDis08,TM_ECTDis_H_DPF_KL,TM_ECTDis_KL,TmEcTpSp_TpEcuCtrRst_P,TmEcTpSp_TpEcuCtrT_P,TmEcTpSp_TpEcuThd0_P,TmEcTpSp_TpEcuThd1_P,TmEcTpSp_TpEcuThd2_P,TmEcTpSp_TpEcuThd3_P,TmEcTpSp_TpEcuThd4_P,TmEcTpSp_TpEcuThd5_P,TmEcTpSp_TpEcuThd6_P,TmEcTpSp_TpEcuThd7_P,TmEcTpSp_TpEcuThd8_P,TmEctSp_StEcuCtlEna_P,FW_TM_CAF_CT_RUIntT,FW_TM_CoolFanRO_ModeLim,FW_TM_DFI_OprMode,FW_TM_RO_ASSStopMode_OnDly,FW_TM_RO_BR_Enable_HI,FW_TM_RO_Err_Fac,FW_TM_RO_FacTCorr2IntIn,FW_TM_RO_IntScal_Sel,FW_TM_RO_ISRD_ECT,FW_TM_RO_ISRD_ECT_TDly,FW_TM_RO_ISRD_ECTHi,FW_TM_RO_ISRD_ECTLo,FW_TM_RO_ISRD_ECTRef,FW_TM_RO_ISRD_ECTsolo,FW_TM_RO_ISRD_EngSpd,FW_TM_RO_ISRD_EngSpd_TDly,FW_TM_RO_ISRD_SenOil,FW_TM_RO_ISRD_SenOilsolo,FW_TM_RO_ISRD_TCor2,FW_TM_RO_ISRD_TMax,FW_TM_RO_Lim,FW_TM_RO_Load_Sel,FW_TM_RO_LoadCalc_Sel,FW_TM_RO_MAFEngSpd_DE,FW_TM_RO_RatHeatInput,FW_TM_RO_UpModDelay,KL_TM_RO_DifEotEct_Pwr_Req,KL_TM_RO_ECTOut,KL_TM_RO_Exh_Temp,KL_TM_RO_ExtAir_Temp3,KL_TM_RO_MAFEngSpdA_U8,KL_TM_RO_MAFEngSpdB_U8,KL_TM_RO_POEngSpd_U8,KL_TM_RO_TCorrection2,KL_TM_RO_TCorrection2a,KL_TM_RO_VehSpd_U16,sst_TM_ECTIn_Plaus2,sst_TM_RO_DifEotEct_Pwr_Req,sst_TM_RO_Eng_Spd2,sst_TM_RO_Eng_Trq,sst_TM_RO_Exh_Temp_Req,sst_TM_RO_ExtAir_Temp2,sst_TM_RO_Inj_FIRate,sst_TM_RO_Inj_VolCyl,sst_TM_RO_MAF2,sst_TM_RO_TCorrection2,sst_TM_RO_TCorrection2a,sst_TM_RO_VSpd,Tm_TDlyEeWr_P,TmHi_FacCor2EeRstThd_P,TmHi_FacLimQhtMemDmdOpgShttr_P,TmHi_FlgIgEngRunMod_P,TmHi_FlgIgSwRunMod_P,TmHi_FlgIniEe_P,TmHi_QInjSel_P,TmHi_StEcuModlEna_P,TmMdl_Fac3Cor2Ee_P,TmMdl_FacTEngShutOf_A,TmMdl_FacTEngShutOf_L,TmMdl_FacTpEcuFanReqAftRun_L,TmMdl_FacTpQhtTchFanReqAftRun_L,TmMdl_FacTpQhtVehFanReqAftRunDpfRgn_L,TmMdl_FacTpQhtVehFanReqAftRunDpfRgnTDly_P,TmMdl_FacTpQhtVehFanReqAftRunDpfRgnX_A,TmMdl_FuInjModSwt_P,TmMdl_StandHeatIntglFac01_L,TmMdl_StandHeatIntglFac0_A,TmMdl_StandHeatIntglFac11_L,TmMdl_StandHeatIntglFac1_A,TmMdl_TpEcuFanReqAftRun_A,TmMdl_TpIntkAirFanReqAftRun_A,TmMdl_TpIntkAirFanReqAftRun_L,TmMdl_TpMaxQhtTch_P,TmMdl_TpQhtTchFanReqAftRun_A,TmMdl_TpTchQhtOfsCor_A,TmMdl_TpTchQhtOfsCor_L,TmClpmp_CnvrLinVoltFac_P,FW_PremAirTmOpen_En,FW_TMVSpdLimH,FW_TMVSpdLimL,FW_TMVSpd_TFiltOff,FW_TMWKR_H_S8,FW_TMWKR_L_S8,FW_TM_EAT_MxH,FW_TM_EAT_MxL,FW_TM_EAT_Mx_Sel,FW_TM_ECT_DrvProg_Dly,FW_TM_ECT_DrvProg_EatHi,FW_TM_ECT_DrvProg_EatLo,FW_TM_ECT_IATH,FW_TM_ECT_IATL,FW_TM_ECT_IAT_EngSpd_Filt,FW_TM_ECT_IAT_TFilt,FW_TM_ECT_IAT_TFiltOff,FW_TM_ECT_OilTH,FW_TM_ECT_OilTL,FW_TM_ECT_OilT_TFiltOff,FW_TM_ECT_Ref_DrvProg,FW_TM_ECT_Ref_EAT,FW_TM_ECT_Ref_GA,FW_TM_ECT_Ref_IAT,FW_TM_ECT_Ref_MnFreezeDly,FW_TM_ECT_Ref_MnFreezeEngSpd,FW_TM_ECT_Ref_OilT,FW_TM_ECT_Ref_PremAir,FW_TM_ECT_Ref_Regen_Lo,FW_TM_ECT_Ref_TGETR,FW_TM_ECT_Ref_TrlrState,FW_TM_ECT_Ref_TROil_1,FW_TM_ECT_Ref_TROil_2,FW_TM_ECT_Ref_VSpd,FW_TM_ECT_Ref_WKR,FW_TM_ECT_Regen_EAT,FW_TM_ECT_Regen_ECTH,FW_TM_ECT_Regen_ECTL,FW_TM_ECT_Regen_EngRun_Dly,FW_TM_ECT_Regen_EngSpd_Hi,FW_TM_ECT_Regen_EngSpd_Lo,FW_TM_ECT_Regen_Freeze_Dly,FW_TM_ECT_TrlrState_EatHi,FW_TM_ECT_TrlrState_EatLo,FW_TM_TGETEnMan,FW_TM_TGETRH,FW_TM_TGETRL,FW_TM_TGETR_TFilt,FW_TM_T_PremAir,FW_TM_WKR_TFilt,FW_TM_WKR_TFiltOff,idx_TmSelVehVarDrvProgRednCoolt,idx_TmSelVehVarTrlrStsRednCoolt,TmEcTpSp_AATEngOilTpEcTpCodn_P,TmEcTpSp_AATEngOilTpEcTpDly2_P,TmEcTpSp_AATEngOilTpEcTpDly_P,TmEcTpSp_AATEngOilTpEcTpLo_P,TmEcTpSp_AATEngOilTpStrtEcTp_P,TmEcTpSp_AATThdLoOilTpEcTpHi_P,TmEcTpSp_AATThdLoOilTpEcTpLo_P,TmEcTpSp_EcTpSpMinAATOilTp_P,TmEcTpSp_EcTpSpMinHiMdlThd_P,TmEcTpSp_EcTpSpMinHiMdl_P,TmEcTpSp_EcTpSpMinShttrPmp1_P,TmEcTpSp_EcTpSpMinShttrPmp2_P,TmEcTpSp_MaskDrvrProg_P,TmEcTpSp_MaskHiPP_P,TmEctSp_MaskPred1_P,TmEctSp_MaskPred_P,TmEctSp_TpPredHi1_P,TmEctSp_TpPredHi2_P,TmEctSp_TpPredHi_P,TmEctSp_TpPredLo1_P,TmEctSp_TpPredLo2_P,TmEctSp_TpPredLo_P,TmPremAirTmOpenGrdtFaiEna_P,TM_ECT_IAT_VehSpd_sst03,TM_EngSpd_sst05,TM_IAT_EngSpd_KL05,TM_IAT_VehSpd_KL03,AdapAltitudeTempCorrV8,EBG_RP_SST,NISTV17,PWV,sst_Baro,SWPEDV16,TL8V08,VCANV05,VCANV08,FW_PremAirTmDirt_En,FW_TMEATLimH,FW_TMEATLimL,FW_TMEATTGetLimH,FW_TMEATTGetLimL,FW_TMTGetLimH,FW_TMTGetLimL,FW_TM_EAT_MnH,FW_TM_EAT_MnL,FW_TM_ECT_PreStrt_TFilt,FW_TM_ECT_Ref_EATLimH,FW_TM_ECT_Ref_EATLimL,FW_TM_ECT_Ref_Lo,FW_TM_ECT_Ref_PremADiagOk_En,FW_TM_ECT_Ref_PreStrt,FW_TM_ECT_Ref_Regen_Prev,FW_TM_PFltRegen_Mode,FW_TM_TS_TROilReq_Lim1,FW_TM_TS_TROilReq_Lim2,FW_TM_T_PremAirDirt,TmEcTpSp_EcTpSpShttrThd_P,TmEcTpSp_SqTcmTpThdSpMax_P,TmEctRef_HdcRefMinDiSt_P,TmPremAirDirtDlyTMax_P,TmPremAirDirtDlyTMin_P,TmPremAirDirtEctThdMaxHi_P,TmPremAirDirtEctThdMaxLo_P,TmTh_NEngPreStrtEctRefLim_P,TmTp_StEnaHybAggr1_P,TmTp_StEnaHybAggr2_P,TmTp_StEnaHybAggr3_P,TmTp_StEnaHybAggr_P,TmTp_StEnaPlgnOpmd1_P,TmTp_StEnaPlgnOpmd2_P,TmTp_StEnaPlgnOpmd3_P,TmTp_StEnaPlgnOpmd_P,TmTp_TDlyStPlgnHybSt1_P,TmTp_TDlyStPlgnHybSt_P,TmTp_THiRefMaxEdrv_P,TmTp_TLoRefMaxEdrv_P,Tm_FlgTpEdrvMask_P,Tm_FlgTpMaxEdrv_P,Tm_LtCcrChAirNEngCorrnFacSp_A,Tm_LtCcrChAirNEngSpFac_A,Tm_LtCcrChAirTpSpCorrn1_M,Tm_LtCcrChAirTpSpCorrnFac2_L,Tm_LtCcrChAirTpSpCorrnFac4_M,Tm_LtCcrChAirTpSpCorrnFac4Xdir_A,Tm_LtCcrChAirTpSpCorrnFac4Ydir_A,Tm_LtCcrChAirTpSpEom_P,Tm_LtCcrChAirTpSpFac1_M,Tm_LtCcrChAirTpSpFac2_M,Tm_LtCcrChAirTpSpFac2Xdir_A,Tm_LtCcrChAirTpSpFac2Ydir_A,Tm_LtCcrChAirTpSpFac3_M,Tm_LtCcrChAirTpSpFac3Xdir_A,Tm_LtCcrChAirTpSpFac3Ydir_A,Tm_LtCcrChAirTpSpMan_P,Tm_LtCcrChAirTpSpManAcvnFlg_P,Tm_LtCcrChAirTqEngCorrnFacSp_A,Tm_LtCcrChAirTqEngSpFac_A,Tm_LtCcrChAirVCorrnFacSp_A,Tm_LtCcrFlgRegActSel_P,Tm_LtCcrTpChAirSpSel_P,Tm_LtCcrTpDcDcSp_P,Tm_LtCcrTpEmInvSp_P,TmLtCcr_ChAirTpSpTFil_P,TmLtCcr_PGasIntk1_P,TmLtCcr_StSeldColdStrt_P,TmLtCcr_StSeldDPFRegn_P,TmLtCcr_StSeldLiOff_P,TmLtCcr_StSeldNormCmb_P,TmLtCcr_StSelHeatgCmbMod_P,TmLtCcr_TpChAir1_M,TmLtCcr_TpChAir1X_A,TmLtCcr_TpChAir1Y_A,TmLtCcr_TpChAir2_M,TmLtCcr_TpChAir2X_A,TmLtCcr_TpChAir2Y_A,TmLtCcr_TpChAirClcdMax_P,TmLtCcr_TpChAirClcdMin_P,TmLtCcr_TpChAirSpDpfFlg_P,TmLtCcr_TpChAirSpDpfMan_P,TmLtCcr_TpChAirSpRgnFlg_P,TmLtCcr_TpColdCmbChmb_P,TmLtCcr_TpEngOil1_P,TmLtCcr_TpEngOilStrt1_P,TmLtCcr_TpGasIntk1_P,TmLtCcr_TpNotColdCmbChmb_P,FW_TM_LimToilEhpOn_Req,FW_TM_RoLimEhpOn_Sw,FW_TM_RoLimToilOn_Sw,Tm_DlyTAftRunCoolgPmp_P,TmPmp_ArTchForQhtMdl_P,TmPmp_BatVoltDiAftRun_P,TmPmp_DeacvtAftRunHvacFlg_P,TmPmp_EctMinTpCtlEwpHeatr_P,TmPmp_EngOilMinTpCtlEwpHeatr_P,TmPmp_FlgRunMod_P,TmPmp_FlgTstrAftRunDeacvd_P,TmPmp_GrdtIntegrQhtTch_P,TmPmp_IdxCodnMdlAcvtAftRunFwd_P,TmPmp_IdxCodnMdlDeacvtAftRun_P,TmPmp_MpExhIdxTch_P,TmPmp_MpExhSelnQTch_P,TmPmp_MpExhSpcCpQTch_P,TmPmp_QBeamTchEmiIdx_P,TmPmp_QTchEngSoErrIninDlyT_P,TmPmp_QTchEngSoTIninFac_L,TmPmp_QTchEngSoTIninFacBpr_A,TmPmp_RunOnTGbOilHiMod_P,TmPmp_ScrcmDosPmpAftRunErrReq,TmPmp_ScrcmDosPmpAftRunMaxReq,TmPmp_ScrcmDosPmpAftRunRelSel,TmPmp_ScrcmDosPmpAftRunSNAReq,TmPmp_StEcuModlEna_P,TmPmp_TDebPmpAftRunCorrn2Dpf_P,TmPmp_TDlyBatVoltDiAftRun_P,TmPmp_TEnaBusOff_P,TmPmp_TFilQhtTchTpFall_P,TmPmp_TFilQhtTchTpRisng_P,TmPmp_THeatrPmpAftRunEnaReq_P,TmPmp_THeatrPmpAftRunReqSeln_P,TmPmp_TMinHeatrPmpAftRunReq_P,TmPmp_TpGbOilLimPmpAftRun_P,TmPmp_TPmpAftRunCorrn2_A,TmPmp_TPmpAftRunCorrn2_L,TmPmp_TPmpAftRunCorrn2a_A,TmPmp_TPmpAftRunCorrn2a_L,TmPmp_TPmpAftRunCorrn2Dpf_L,TmPmp_TPmpAftRunCorrn2DpfX_A,TmPmp_TPmpAftRunEcTp_A,TmPmp_TPmpAftRunEcTp_L,TmPmp_TPmpAftRunQhtTch1_L,TmPmp_TPmpAftRunQhtTch_A,TmPmp_TPmpAftRunQhtTch_L,TmPmp_TPmpEnaLim_P,TmPmp_TpQhtTchTpMax_P,TmPmp_TrbMinTpCtlEwpHeatr_P,TmPmp_VAirFlowFanQTrf_A,TmPmp_VAirFlowQTrf_M,TmPmp_VAirFlowVehVQTrf_A,TmClpmp_AcvnFlgDispEcu_P,TmDispEcu_Em2CoolReqSqMax_P,TmDispEcu_Em2CoolReqSqMin_P,TmDispEcu_Em2CoolReqThdErr_P,TmDispEcu_Em2CoolReqThdErrSub_P,TmDispEcu_MaskEngCoolgSysErr_P,TmDispEcu_MaskEngCoolgSysFlt_P,TmDispEcu_TDlySysErr_P,FW_TM_CP_ASSStopMode_en,FW_TM_CP_ASSStopMode_OffDly,TmClpmp_Bms48StCntctrD_P,TmClpmp_CtlHvacPwmSqMin_P,TmClpmp_EcuAftRunDlyT_P,TmClpmp_EcuOnReqAcvFlg1_P,TmClpmp_ElPmpErrModPwm_P,TmClpmp_EnaFlgDryRunAcvn_P,TmClpmp_EngClpmpLinReqPwmThd_P,TmClpmp_EngPmpAcvMan_P,TmClpmp_EngPmpInvFlg_P,TmClpmp_EngPmpPwmMan_P,TmClpmp_EngPostRunAcvDlyT_P,TmClpmp_EngSwModPwmLimMax_P,TmClpmp_EpdElPwrLimdMax_A,TmClpmp_EpdElPwrLimdMax_L,TmClpmp_FlgEcmLin2AcvnReqTDly_P,TmClpmp_LinAcvnMask_P,TmClpmp_LinAcvnPmpPn48VSq_P,TmClpmp_LinAcvnPmpPn48V_P,TmClpmp_LinAcvnPn48VoltSq_P,TmClpmp_LinAcvnPn48Volt_P,TmClpmp_LinAcvnPn48VSq_P,TmClpmp_LinAcvnPn48V_P,TmClpmp_LinAcvnStCntctrD_P,TmClpmp_LinDeacvnPmpPn48VSq_P,TmClpmp_LinDeacvnPmpPn48V_P,TmClpmp_LinDeacvnPn48VoltSq_P,TmClpmp_LinDeacvnPn48V_P,TmClpmp_LinDeacvnStCntctrD_P,TmClpmp_LinEnaAcvFlgMed_P,TmClpmp_LinEnaAcvFlg_P,TmClpmp_LinMedManAcvFlg_P,TmClpmp_MrgLin2AcvnFlg_P,TmClpmp_PercAftRunDeacvn_P,TmClpmp_PercAftRunPerc_L__2,TmClpmp_PercAftRunTBpr_A__2,TmClpmp_PercDryRun_P,TmClpmp_ReqFltModFlgPwm_P,TmClpmp_StEcuLinAcv_P,TmClpmp_TDlyIgSwRunOff_P,TmClpmp_TIniSetDryRun_P,TmPmp_EngClpmpEmmoOffSt2_P,TmPmp_EngClpmpEmmoOffSt_P,TmPmp_EngClpmpPostRunAcvT2_P,TmPmp_EngClpmpPostRunAcvT_P,TmPmp_HdcSt_P,flg_TmHtCcrVlvAgrReqInv_P,flg_TmHtCcrVlvAgrReqMan_P,flg_TmHtCcrVlvAgrReqRels_P,flg_TmLtHtCcrVlvFanAcv_P,flg_TmLtHtCcrVlvReqAcv_P,flg_TmLtHtCcrVlvReqEwpMan_P,flg_TmLtHtCcrVlvReqMan_P,FW_TM_ERRECT_en,FW_TM_ErrEctLow_en,FW_TM_ErrECTPos,FW_TM_HV_AC_Pulse_en,FW_TM_HV_Err_Config,FW_TM_HVECT_Delay,FW_TM_HVECT_H,FW_TM_HVECT_L,FW_TM_HVECT_Pulse,FW_TM_HVECT_Pulse_TOff,FW_TM_HVECTLow,FW_TM_HVFFDly_en,FW_TM_HVFFMode_en,FW_TM_HVMalfMode_en,FW_TM_HVNIST_H,FW_TM_HVNIST_L,FW_TM_HVNIST_SC,FW_TM_HVPulse_EATMax,FW_TM_HVPulse_ECTMax,FW_TM_HVPulse_ECTMin,FW_TM_HVPulse_En,FW_TM_HVPulse_T,FW_TM_HVPulse_T2,FW_TM_HVPulse_TPer,FW_TM_HVPulse_TPer2,FW_TM_HVPulse_TRun,FW_TM_HVReq,FW_TM_HVReq_Delay,FW_TM_HVTCloseMx,FW_TM_HVUBAT_H,FW_TM_HVUBAT_L,FW_TM_HVUBAT_TFilt,FW_TM_lowEctPos,FW_TM_RotVEngRunMode,FW_TM_RotVEngRunMode_RO,FW_TM_RotVInvert,FW_TM_RotVlvMalf_Cntl,FW_TM_RotVlvMalf_Cntl_en,FW_TM_TplsPer,FW_TM_Tplstime,FW_TM_TplsVal,FW_TMManHV,FW_TMManHV_en,FW_TMManRotV,FW_TMManRotV_en,idx_TmHtCcrVlvAgrDfiReq_P,idx_TmLtHtCcrVlvReqBR_P,idx_TmLtHtCcrVlvReqRelsBR_P,idx_TmPumpRunOnReqBR_P,n_TmHtCcrVlvAgrNEng_P,perc_TmHtCcrVlvAgrEgr_P,perc_TmHtCcrVlvAgrLoaEng_P,t_TmHtCcrVlvAgrDlyCls_P,t_TmHtCcrVlvAgrDlyOpend_P,t_TmLtHtCcrVlvEngRunDly_P,t_TmLtHtCcrVlvEngRunTmr_P,TM_ECTOut04,TM_RotVLim_KL,TmCcr_StEcuCoolgCnvrEna_P,TmHeatrVlv_RunOnAatTpThd_P,TmHeatrVlv_RunOnEctTpTDly_P,TmHeatrVlv_RunOnEctTpThd_P,TmHeatrVlv_RunOnQhtCorThd_P,TmHeatrVlv_RunOnTDly_P,TmHeatrVlv_RunOnTpQhtTchThd_P,TmTh_AcvThDiagAcvnFlg_P,TmTh_AcvThDiagPosn_P,TmTh_FailSafePosnMin_P,TmTh_LimDiagcLoPercOff_P,TmTh_LimDiagcLoPercOn_P,TmTh_LimDiagcPercFlg_P,TmTh_LimDiagcPercMax_P,TmTh_LimDiagcUpPercOff_P,TmTh_LimDiagcUpPercOn_P,TmTh_LimThReqTpFlg_P,TmTh_LimThThdAATHi_P,TmTh_LimThThdAATLo_P,TmTh_PercThPremAirStop_P,TmTh_PosnRotVlvPmpErrMod_P,TmTh_RsgRunOnAcvnFlg_P,TmTh_RsgRunOnClpmpAcvnThdPerc_P,TmTh_RsgRunOnPercReq_P,TmVlv_FlgHwCptHeatrVlvSwtEna_P,TmVlv_FlgHwCptHtLtVlvSwtEna_P,tp_TmCooltHtToLtHtCcrVlvAct_P,FW_TM_CCR_StuckChck_ECT_Ref,FW_TM_CCR_StuckChck_ECTRef_T,FW_TM_CCR_StuckChck_Min_Delta,FW_TM_CCR_StuckChck_Time,FW_TM_CCRTR_AddCntr,FW_TM_CCRTR_AddMx,FW_TM_CCRTR_AddVal,FW_TM_CCRTR_AvgCntr,FW_TM_CCRTR_ECTHi,FW_TM_CCRTR_ECTLo,FW_TM_CCRTR_ECTRef,FW_TM_CCRTR_TCMHi,FW_TM_CCRTR_TCMLo,FW_TM_CCRTRTCM_Eskal_Lo,FW_TM_CCRTRTCMHi_Eskal_Hi,FW_TM_CCTTR_ECT_Lim,FW_TM_ECT_Ref_Hi,FW_TM_GA_EAT_Lim,FW_TM_MNMX_ECTMx,FW_TM_MNMX_ECTStrt,FW_TM_MNMX_ECTTDly,FW_TM_MNMX_ECTTimerStrt,FW_TM_MNMX_GA_en,FW_TM_MNMXOfs,FW_TMCCConfig,FW_TMCCECTDelta,FW_TMCCECTDeltaT,FW_TMCCGRDTime,FW_TMCCPos,FW_TMCCRECTOfs_en,FW_TMCCRTPwrFilt,FW_TMCCT_HV_Open_Del,FW_TMCCT_Stuck_Check_en,FW_TMCCTEATLim_Hi,FW_TMCCTEATLim_Lo,FW_TMCCTECTLim_EngSpd_en,FW_TMCCTECTLim_Hi,FW_TMCCTECTLim_Lo,FW_TMCCTEngSpdLim_en,FW_TMCCTEngSpdLim_en_Tdly,FW_TMCCTHV,FW_TMCCTHV_en,FW_TMCCTimeFacErr,FW_TMCCTimeMNHi,FW_TMCCTimeMNLo,FW_TMCCTimeMXHi,FW_TMCCTimeMXLo,FW_TMCCTRefLim,FW_TMGAIniDelay,FW_TMGAPos1,FW_TMGAPos1_HT,FW_TMGAPos2,FW_TMGAPos2_HT,FW_TMGAPos3,FW_TMGAPos3_HT,FW_TMGAPremAirDi_P,FW_TMMODECT_Sel,FW_TMPCTDelay,FW_TMPCTEATLim,FW_TMPCTECT_Sel,FW_TMPCTECTRef_Dis,FW_TMPCTMan,FW_TMPCTMan_En,FW_TMPreCTMan,FW_TMPreCTMan_En,FW_TMThrustDeltaLim,FW_TMThrustECTSel,FW_TMThrustEngSpd,FW_TMThrustHi_en,FW_TMThrustLim,FW_TMThrustLT,FW_TMThrustTime,FW_TMThrustVsp,KL_TM_CCRCTPreDelayT,sst_TM_CCRPreDiffEctRef,ThCtlPercPremAirMin_P,ThCtlTPremAirFrmAcv_A,ThCtlTPremAirFrmAcv_L,TM_CCR_ECT_Jal_02,TM_CCR_ECT_MNMX08,TM_CCR_ECTJal_KL,TM_CCR_ECTOfs_VS_PW_33,TM_CCR_EngPwrInd_03,TM_CCR_ExtAirMNMX04,TM_CCR_MNMXCT_KF,TM_CCR_PCTEAT_KFS8,TM_CCR_VS_03,TM_ECTDelta08,TM_ExtAirTemp04,TM_ExtAirTemp08,TM_ThrustEAT_KL,TmCcrCtlr_StEcuEna_P,TmTh_EcTpDplAAT_A,TmTh_EcTpDplAATClm_M,TmTh_EcTpDplClm_A,TmTh_EcTpPoutpSeln_P,TmTh_PercPoutpEctLo_M,TmTh_PercPoutpEctLoX_A,TmTh_PercPoutpEctLoY_A,TmTh_PercPoutpEctMid_M,TmTh_PercPoutpEctMidX_A,TmTh_PercPoutpEctMidY_A,TmTh_SelnTpThdHi_P,TmTh_SelnTpThdLo_P,FW_TMTSollHi,FW_TMTSollLo,EngOilTp_SqAmbAirTpErr_P,EngOilTpMdl_FacEngTqCodn_L,EngOilTpMdl_FacLoTpHiPCodn_P,EngOilTpMdl_FacLoTpLoPCodn_P,EngOilTpMdl_HeatgEcTpThd_P,EngOilTpMdl_OfsEcTpCodn_L,EngOilTpMdl_OfsHeatgEcTpGrdtF_P,EngOilTpMdl_OfsHeatgEcTpTDly_P,EngOilTpMdl_OfsHeatgEcTpTGrdt_P,EngOilTpMdl_OfsHeatgEcTpThd_P,EngOilTpMdl_OfsTpOilPmp2_L,EngOilTpMdl_SqEcTOutErr_P,EngOilTpMdl_SqInin_P,EngOilTpMdl_SqVehVErr_P,FW_TOIL_CCPT_ECT_H,FW_TOIL_CCPT_ECT_L,FW_TOIL_CCPT_EngSpd,FW_TOIL_CCPT_RotVlv,FW_TOIL_CCPT_T_RotVlv_Dly_Hi,FW_TOIL_CCPT_T_RotVlv_Dly_Lo,FW_TOIL_CHS_en,FW_TOIL_CHS_Sel,FW_TOIL_CHSDeltaLim,FW_TOIL_CHSECTLim,FW_TOIL_CHST_MX,FW_TOIL_Config,FW_TOIL_CRLC_AktDly,FW_TOIL_CRLC_TIME,FW_TOIL_Eng_Run_Mode_Sw,FW_TOIL_Err_Config,FW_TOIL_Err_TDelay,FW_TOIL_FAC_CRLC_CCPH,FW_TOIL_FAC_CRLC_CCPT,FW_TOIL_FAC_CRLC_HTHP,FW_TOIL_FAC_CRLC_HTLP,FW_TOIL_FAC_CRLC_LTHP,FW_TOIL_FAC_CRLC_LTLP,FW_TOIL_FAC_OilPSw_Dly,FW_TOIL_FAC_OilPSw_Hi,FW_TOIL_FAC_OilPSw_Lo,FW_TOIL_FAC_OilPSw_T,FW_TOil_Fac_VS_EAT,FW_TOIL_FAC_WaPu_en,FW_TOIL_GRD_TIME_L,FW_TOIL_H_MX,FW_TOIL_HEATUP_ECT_Mn,FW_TOIL_IgnPwf_en,FW_TOIL_IK,FW_TOIL_IMN,FW_TOIL_IMX,FW_TOIL_InitDelayCAN,FW_TOIL_InitDelayMax,FW_TOIL_L_GRD_MX,FW_TOIL_LPF,FW_TOIL_ManCHS,FW_TOIL_OFS_VSShuttr_Disable,FW_TOIL_SenOilTemp_Grad_Hi,FW_TOIL_SenOilTemp_Grad_Lo,FW_TOIL_SenToilGrad_DelayTime,FW_TOIL_Sw_TAST,KF_TOIL_FAC_ECT_TAST,KL_TOIL_FAC_WaPu,KL_TOIL_OFS_ECT,KL_TOIL_Stop_Time,sst_TOIL_ECT,sst_TOIL_FAC_WaPu,sst_TOIL_Stop_Time,sst_TOIL_TAST_08,TmOilTpMdl_AcvnSelnFlg_P,TmOilTpMdl_HdcCodnSt_P,TmOilTpMdl_HybSt1_P,TmOilTpMdl_HybSt2_P,TmOilTpMdl_SysIniTOnDly_P,TOIL_CHS_KF,TOIL_EAT_04,TOIL_EAT_08,TOIL_ECT_08,TOIL_ESOT_08,TOIL_ESOT_KL,TOIL_FAC_NIST_KL,TOIL_FAC_TRQ_KL,TOIL_Fan_03,TOIL_HI_ECTFAC_KL_08,TOIL_NIST_08,TOIL_OFS_NIST_LOAD_KF_88,TOIL_OFS_NIST_LOAD_KF_Cod_88,TOIL_OFS_NIST_OILPSW_KL_08,TOIL_OFS_VS_EAT_KF_84,TOIL_OFS_VS_Fan_KF,TOIL_OFS_VS_TOil_KF_33,TOIL_TOil_03,TOIL_TRQ2_08,TOIL_TRQ_08,TOIL_VS_03,TOIL_VS_04,TOIL_VS_08,FW_TMFATime1,FW_TMFATime2,FW_TMFATimeLim1,FW_TMFATimeLim2,FW_TMFA_en,FW_TMGAConfig,FW_TMGAConTime,FW_TMGAConTimeEng,FW_TMGAECTLim_Cond,FW_TMGAECTLim_Start,FW_TMGAMan,FW_TMGAManHi,FW_TMGAManLo,FW_TMGAManMid,FW_TMGAMan_act,FW_TMGANmotH,FW_TMGANmotL,FW_TMGATime1,FW_TMGATime2,FW_TMGATime3,FW_TMGATimeWait,FW_TMGAVspdH,FW_TMGAVspdL,FW_TMGA_EATLimH,FW_TMGA_EATLimL,FW_TMGA_MLH,FW_TMGA_MLL,FW_TMTSollMid,TmCcrCt_StsThAdpnErrEna_P,TmCcr_StEcuCcrCtEna_P,TmTh_FlgIgOnCtlDeacvnThGovr_P,TmTh_PremairChkFlgAdpnDeacvn_P,TM_CCRFATime08,TM_CCRFATime_KL,TM_CCRGADEAT06,TM_CCRGAEAT04,TM_CCRGAEAT_KF,TM_CCRGA_EAT08,TM_CCRGA_EAT_KL,Epd_ClpmpCoolgReqBpr_A,Epd_ClpmpCoolReqFac_L,Epd_ClpmpMinVoltFacBpr_A,Epd_ClpmpMinVoltFac_L,Epd_ClpmpPmaxAllwd_P,Epd_EbstrMinCurAllwd_P,Epd_EbstrMinVoltFacBpr_A,Epd_EbstrMinVoltFac_L,Epd_PwrMax48VManReq_P,Epd_PwrMax48VManVal_P,Tm_AmbAirPDft_P,Tm_AmbAirTpSqThd_P,Tm_EngOilPManReq_P__2,Tm_EngOilPManReqFlg_P,Tm_EngOilPOffSet_P,Tm_EngOilPReqDifFac_P,Tm_EngOilSqThd_P,Tm_NEngOilPmp_A,Tm_NEngOilPmpLo_A,Tm_NEngOilPmpMid_A,Tm_PcdEnaFlgPwmDith_P,Tm_PcdIntgNThdOff_P,Tm_PcdIntgNThdOn_P,Tm_PcdIvsFlg_P,Tm_PcdIvsPwmFlg_P,Tm_PcdOilTpFltEnaThd_P,Tm_PcdOilTpFltEnaThdLo_P,Tm_PcdOilTpHysDifHi_P,Tm_PcdOilTpHysDifLo_P,Tm_PcdOilTpHysHi_P,Tm_PcdOilTpHysLo_P,Tm_PcdOilTpMinEna_P,Tm_PcdOilTpThdHiOff_P,Tm_PcdOilTpThdHiOn_P,Tm_PcdOilTpThdOff_P,Tm_PcdOilTpThdOn_P,Tm_PcdPreCtlPReq_A,Tm_PcdPwmDithHiCt_P,Tm_PcdPwmDithPerdCt_P,Tm_PcdTpOilSel_P,Tm_PEngOilDft_P,Tm_POilDmd1_M__2,Tm_POilDmd1Lo_M,Tm_POilDmd1Mid_M,Tm_TpOilDft_P,Tm_TpOilSqThd_P,Tm_TqEngOilPmp_A,Tm_TqEngOilPmpLo_A,Tm_TqEngOilPmpMid_A,TmPcd_CamsftAbsvSumTFil_P,TmPcd_CamsftDifMaxAg_P,TmPcd_EnaPistCoolgRunT_L,TmPcd_EnaPistCoolgRunTBpr_A,TmPcd_EngNManThd_P,TmPcd_EngOilHiPReqEnaFlg_P,TmPcd_EngOilPMaxLim_P,TmPcd_EngOilPReqThd_P,TmPcd_EngStManChk_P,TmPcd_ErrSaveEnaFlg_P,TmPcd_FacICtlOilPErr_P,TmPcd_FacICtlOilPmpReq_M,TmPcd_FacICtlOilPmpReqPost_L,TmPcd_FacPCtlOilPmpReq_M,TmPcd_FacPwmICtlOilPmpReq_M,TmPcd_FacPwmICtlOilPmpReqX_A,TmPcd_FacPwmICtlOilPmpReqY_A,TmPcd_FlgEnaEngStChk_P,TmPcd_FlgICtlZeroRunRstEna2_P,TmPcd_FlgOilPmpReqManEna_P,TmPcd_FlgPOilPwmPreCtlSeln_P,TmPcd_FlgTDlyAcvnAcv_P,TmPcd_InjSwtOffEnaFlg_P,TmPcd_ManSwtStN_P,TmPcd_MaskEngStEna_P,TmPcd_MaskEom_P,TmPcd_NEngPmpReqRstAcv_P,TmPcd_NEngPmpReqRstLim_P,TmPcd_NEngPwmPreCtlOilPmp_A,TmPcd_NMotMinPOilStrt_P,TmPcd_OilPmpPercReqSwt_P,TmPcd_OilPNotVldCtThd_P,TmPcd_OilPRelFac_P,TmPcd_OilTpMin_P,TmPcd_OilTpThd_P,TmPcd_OilTpThdMax_P,TmPcd_PEngOilRelFildDifFall_P,TmPcd_PEngOilRelFildDifRisng_P,TmPcd_PICtlZeroRunRstErrMax_P,TmPcd_PICtlZeroRunRstErrMin_P,TmPcd_POilErrICtlFac_A,TmPcd_POilErrPCtlFac_A,TmPcd_POilPmpReqRstLim_P,TmPcd_POilRelThd_P,TmPcd_POilStrtDi_P,TmPcd_POilStrtMin_L,TmPcd_POilStrtMinX_A,TmPcd_PwmFacICtlOilPmpReqRaw_P,TmPcd_PwmICtlOilPmpReqMax_P__2,TmPcd_PwmICtlOilPmpReqMin_P__2,TmPcd_PwmICtlOilPmpReqRst_P__2,TmPcd_PwmOilPmpReqDi_P,TmPcd_PwmOilPmpReqDith_P,TmPcd_PwmOilPmpReqDithOfs_L,TmPcd_PwmOilPmpReqDithOfsX_A,TmPcd_PwmOilPmpReqEnaKm_P,TmPcd_PwmOilPmpReqEnaKmFlg_P,TmPcd_PwmOilPmpReqMan_P,TmPcd_PwmOilPmpReqMax_P,TmPcd_PwmOilPmpReqMin_P,TmPcd_PwmOilPmpReqMinStrt_P,TmPcd_PwmOilPmpReqStrt_P,TmPcd_PwmPCCorOffOilPmpReq_P,TmPcd_PwmPCCorOnOilPmpReq_P,TmPcd_PwmPICtlOilPmpReqMax_P,TmPcd_PwmPICtlOilPmpReqMin_P,TmPcd_PwmPreCtlNTpOilPmpReq_M,TmPcd_PwmPreCtlOilPmpReqFall_M,TmPcd_PwmPreCtlOilPmpReqRisng_M,TmPcd_StEcuEna_P,TmPcd_TDlyAcvnTSoTpOil_M,TmPcd_TDlyAcvnTSoTpOilX_A,TmPcd_TDlyAcvnTSoTpOilY_A,TmPcd_TDlyEngOilPReq_P,TmPcd_TDlyErrEntry_P,TmPcd_TDlyPOilRel_P,TmPcd_TEngOilRelFild_P,TmPcd_TEngOilRelFildDly_P,TmPcd_TFildPCCorOffOilPmpReq_P,TmPcd_TFildPCCorOnOilPmpReq_P,TmPcd_TICtlOilPmpReqFild_P,TmPcd_TIniOilPNotVldCtr_P,TmPcd_TLoPOilPmpReqRstDly1_P,TmPcd_TmOilPCtlDifErrThd_P,TmPcd_TpOilICtlFac_A,TmPcd_TpOilPCtlFac_A,TmPcd_TpOilPwmPreCtlOilPmp_A,TmPcd_TpOilPwmPreCtlPmpReq_A,TmPcdLrng_EngNThd_P,TmPcdLrng_FlgEna_P,TmPcdLrng_PEngOilReqChgMax_P,TmPcdLrng_PEngOilReqLim_P,TmPcdLrng_PwmICtlChgMax_P,TmPcdLrng_PwmLrndChgMax_P,TmPcdLrng_PwmLrndValMax_P,TmPcdLrng_PwmLrndValMin_P,TmPcdLrng_TDlyEngRunMod_P,TmPcdLrng_TEngOilPReq_P,TmPcdLrng_TEngOilReqDifOk_P,TmPcdLrng_TLrnPwmFil_P,TmPcdLrng_TLrnPwmFilDly_P,TmPcdLrng_TPwmICtl_P,TmPcdLrng_TPwmICtlDifOk_P,FW_ECU_RunOn_activation,FW_TM_OffDlyIgnSwRunMod,Tm_EcuRunOnAcvn2St_P,Tm_EcuRunOnReqSoDebT_P  EnableBusSupport=off
  term_ACComprOff_FanMalf : Terminator
  term_AC_HtrVlv_Front_Plaus_Req : Terminator
  term_AC_HtrVlv_Front_Plaus_ReqSq : Terminator
  term_AC_MAF_Req : Terminator
  term_ClpmpRsg_AftRunReqSt : Terminator
  term_ClpmpRsg_NReq : Terminator
  term_Cod_Func_SGStrat : Terminator
  term_Com_HPP_DrvProgSq : Terminator
  term_CoolFan_MAF_Req : Terminator
  term_CoolFan_Pwr_Req : Terminator
  term_CoolFan_Pwr_Req_RunOn : Terminator
  term_CoolFan_Pwr_Req_RunOn_Ok : Terminator
  term_CoolPump_Mode_Req : Terminator
  term_CoolPump_TCM_Mode_Req : Terminator
  term_CrkcsEvapn_FlgDaiLimEvap : Terminator
  term_CylBank1_FIRate_Rel : Terminator
  term_CylBank2_FIRate_Rel : Terminator
  term_DiagcTstr_EngClpmpActSpd : Terminator
  term_Diagc_FlgNEngMinMaxReq12 : Terminator
  term_Diagc_NEngMinMaxReq12 : Terminator
  term_Diagc_StPrioReq12 : Terminator
  term_Diagc_StWpReq12 : Terminator
  term_Diagc_TqMaxReq12 : Terminator
  term_Diagc_TqMinReq12 : Terminator
  term_Diagc_TqOptmReq12 : Terminator
  term_Dpf_FlgRgnReq : Terminator
  term_ECF_PwrReq_Plaus : Terminator
  term_ECTOut_Raw : Terminator
  term_ECU_RunOn_CoolFan_Req : Terminator
  term_ECU_RunOn_LinShuttr_Req : Terminator
  term_EGR_VlvPos : Terminator
  term_EGR_VlvPos_Err_Mode : Terminator
  term_EcmTm_FlgEngCoolgSysErr : Terminator
  term_EgrVlv2Posn : Terminator
  term_EngSys_PGasIntkAry : Terminator
  term_EngSys_QInjAry : Terminator
  term_EngSys_TpEngAry : Terminator
  term_EngSys_TpEngStrtAry : Terminator
  term_EngSys_TpGasIntkAry : Terminator
  term_Eng_PercIntFanReq : Terminator
  term_EomRampCo_StEomActDes : Terminator
  term_Epd_ClpmpMaxElPwr : Terminator
  term_Epd_EbstrMaxElPwr : Terminator
  term_Epd_PN48EcmMaxAllwdCur : Terminator
  term_Epd_PN48EcmSumElPwr : Terminator
  term_Epd_PwrMax48VRecupEzv : Terminator
  term_ErrEntry_EltFanMalfErr : Terminator
  term_ErrEntry_EltShttrMalfErr : Terminator
  term_ErrEntry_Koch : Terminator
  term_Err_ECTOut_Mode : Terminator
  term_Err_Eng_Spd_Mode : Terminator
  term_Err_IntkAir_Temp_Mode : Terminator
  term_EtdRgn_TpLoCcrDmd : Terminator
  term_Exh_Air_FlowFlt : Terminator
  term_ExtAir_Temp_Mod_SNA_Mode : Terminator
  term_FIRate_Fuel : Terminator
  term_FIRate_Trq : Terminator
  term_FanMalf_Mode : Terminator
  term_FanMalf_Mode_LIN : Terminator
  term_FanMalf_Mode_LINSq : Terminator
  term_FuTpMdl : Terminator
  term_Fu_TpInjrTip : Terminator
  term_HtrVlvMalf_Mode : Terminator
  term_HtrVlv_Mode_Req : Terminator
  term_HtrVlv_State : Terminator
  term_Inj_VolCyl : Terminator
  term_IntkAir_Temp2 : Terminator
  term_LIN_CP_ECP4TransVoltSq : Terminator
  term_LIN_CP_ECP4WakeupStatSq : Terminator
  term_LRS_Mode : Terminator
  term_LTVlv_Mode_Req : Terminator
  term_NetCoorr_FlgEcmLin2AcvnReq : Terminator
  term_Net_Eboost_CoolMassFlow : Terminator
  term_Net_Eboost_CurrLim : Terminator
  term_O2S_Ctrl2_Mode : Terminator
  term_O2SnsrFac2 : Terminator
  term_OilPump_SwitchState : Terminator
  term_OilTemp_Mode : Terminator
  term_RailDiag_EnaFlg : Terminator
  term_RelLoad_OvrHtgPrvn : Terminator
  term_RelLoad_OvrHtgPrvn_Mode : Terminator
  term_SCR_DPDV_tUDosVlvPstFlt1 : Terminator
  term_SenDiagHdr2 : Terminator
  term_SenDiagLamSon2Unplaus : Terminator
  term_SenDiagSensSigErr2 : Terminator
  term_Sen_Oil_Temp2 : Terminator
  term_Sen_Oil_Temp2_SNA_Mode : Terminator
  term_Sen_Oil_Temp_Init_Mode : Terminator
  term_Sen_Oil_Temp_SNA_Mode : Terminator
  term_Sen_Oil_Temp_Sq : Terminator
  term_ShuttrMalf_Mode : Terminator
  term_Shuttr_Pos_Mode : Terminator
  term_Shuttr_Pos_Req : Terminator
  term_Sppl_TpCmprOutMdl2 : Terminator
  term_TM_ASSStopMode_OffDly : Terminator
  term_TM_AddWtrPmp_On_Req : Terminator
  term_TM_CAF_CT_ECT_H : Terminator
  term_TM_CAF_CT_ECT_L : Terminator
  term_TM_CAF_CT_ECU_Temp_Req : Terminator
  term_TM_CAF_CT_Exh_Temp_Req2 : Terminator
  term_TM_CAF_CT_FanLoadInc_Req : Terminator
  term_TM_CAF_CT_Fuel_Temp_Req : Terminator
  term_TM_CAF_CT_HI_Req : Terminator
  term_TM_CAF_Cod_TM_FC_Bit0 : Terminator
  term_TM_CAF_Max_Req_Stop : Terminator
  term_TM_CAF_TR_EnC2 : Terminator
  term_TM_CAF_TR_TGET_Req : Terminator
  term_TM_CAF_VL_elViscoFan_Mode : Terminator
  term_TM_CCRCTExtAir_Temp : Terminator
  term_TM_CCRCT_HV_Open : Terminator
  term_TM_CCRGAEATHi : Terminator
  term_TM_CCRGAEATLo : Terminator
  term_TM_CCRGAEATMid : Terminator
  term_TM_CCRGAStep : Terminator
  term_TM_CCRGA_Hi : Terminator
  term_TM_CCRGA_Hi_out : Terminator
  term_TM_CCRGA_Lo : Terminator
  term_TM_CCRGA_Lo_out : Terminator
  term_TM_CCRGA_Mid : Terminator
  term_TM_CCRGA_Mid_out : Terminator
  term_TM_CCRGA_Req_MNMXDis : Terminator
  term_TM_CCRGA_Req_RefLo : Terminator
  term_TM_CCRGA_act : Terminator
  term_TM_CCRTSHi_act : Terminator
  term_TM_CCRTSLo_act : Terminator
  term_TM_CCRTSMid_act : Terminator
  term_TM_CP_CTR_AC : Terminator
  term_TM_CP_Req_PWM : Terminator
  term_TM_CoolFanPwrReq_Lim : Terminator
  term_TM_CoolFanPwrReq_elVisco : Terminator
  term_TM_CoolFan_RO_Mode : Terminator
  term_TM_CoolFan_RO_Mode_Req : Terminator
  term_TM_ECF_DPFPwrReq : Terminator
  term_TM_ECF_DPFPwrReqMan : Terminator
  term_TM_ECF_LTCrct_Req_ECC : Terminator
  term_TM_ECF_SFT_Req : Terminator
  term_TM_ECT_Ref_Cntr_HT : Terminator
  term_TM_ECT_Ref_Cntr_LT : Terminator
  term_TM_ECT_Ref_Mn_Freeze : Terminator
  term_TM_ECT_Ref_Mn_Load : Terminator
  term_TM_ECT_Ref_Mn_en : Terminator
  term_TM_ECT_Ref_Mx : Terminator
  term_TM_ECT_Ref_PremADiagOk : Terminator
  term_TM_Eng_Pwr_Ind : Terminator
  term_TM_Eng_Run_Mode : Terminator
  term_TM_Eng_Run_Mode_Stop : Terminator
  term_TM_ISRD_Req : Terminator
  term_TM_IgnSwStrtr_Mode : Terminator
  term_TM_LTCoolPump_RunTime6 : Terminator
  term_TM_PC_Req : Terminator
  term_TM_PFltRegenDemand_Mode : Terminator
  term_TM_RO_TCorrection2 : Terminator
  term_TM_RO_curHL : Terminator
  term_TM_RotV_LimPos : Terminator
  term_TM_RotV_Ref : Terminator
  term_TM_ShttrDeIcing_ECTRef : Terminator
  term_TM_Shttr_TjaErrIrrv : Terminator
  term_TM_StopDsabl_Mode : Terminator
  term_TM_TROil_ECTRef : Terminator
  term_TM_TROil_ECTRefVlv : Terminator
  term_TM_TrsmWtrPmp_On_Req : Terminator
  term_TM_idxTmInCpc : Terminator
  term_TOIL_Sensor_dis : Terminator
  term_TOil_Mdl_Int_Out : Terminator
  term_TOil_ShutOff : Terminator
  term_TmBms_EcuRunOnReqFlg : Terminator
  term_TmClpmpErr_ErrSig : Terminator
  term_TmClpmp_ActlElVolt : Terminator
  term_TmClpmp_BlkErrSym : Terminator
  term_TmClpmp_DryRunErrSym : Terminator
  term_TmClpmp_Ecp4ComErrMsgLost : Terminator
  term_TmClpmp_EcuOnReqFlg : Terminator
  term_TmClpmp_ElPmpErrMod : Terminator
  term_TmClpmp_EltErrSym : Terminator
  term_TmClpmp_ErrModIrrvFlg : Terminator
  term_TmClpmp_OverCurErrSym : Terminator
  term_TmClpmp_PmpCtlRawPwm : Terminator
  term_TmClpmp_ReqFltModFlg : Terminator
  term_TmClpmp_VoltErrSym : Terminator
  term_TmEcTpSp_CtrEcuTp{0..9} (10 alike) : Terminator
  term_TmEcTpSp_TpEcuCtrDiRam : Terminator
  term_TmFan_DiagAcvFlg : Terminator
  term_TmFan_FlgCooltReq : Terminator
  term_TmFan_PrevnSmkFmtAftRunFlg : Terminator
  term_TmHeatrVlv_EcuRunOnReqFlg : Terminator
  term_TmHi_FacTCor2Ee : Terminator
  term_TmHi_FacTCor2EeRead : Terminator
  term_TmLtCcr_CacTp : Terminator
  term_TmLtCcr_CacTpSq : Terminator
  term_TmPcdLrng_CtlrFctCoefY100 : Terminator
  term_TmPcdLrng_CtlrFctCoefY20 : Terminator
  term_TmPcd_EepromPDeacvnOdoS : Terminator
  term_TmPcd_PwmOilPmpReq : Terminator
  term_TmPmpLtCcr_EcuRunOnReqFlg : Terminator
  term_TmPmp_ClpmpHiNErrFlg : Terminator
  term_TmPmp_ClpmpLoNErrFlg : Terminator
  term_TmPmp_EngClpmpEMOoff : Terminator
  term_TmPmp_EngClpmpLinReqPwmCoorr : Terminator
  term_TmPmp_FlgChrgrEwpHeatrReq : Terminator
  term_TmPmp_RsgCcrEcuRunOnReqFlg : Terminator
  term_TmPmp_THeatrPmpAftRunReq1 : Terminator
  term_TmPmp_THeatrPmpAftRunReq6 : Terminator
  term_TmPmp_TpQhtTch : Terminator
  term_TmPmp_TpQhtTchDram : Terminator
  term_TmReqMinPremAirDirtFlag : Terminator
  term_TmRsvBms_EcuRunOnReqFlg : Terminator
  term_TmRsvLtCcr_EcuRunOnReqFlg : Terminator
  term_TmSigIf_StEcu : Terminator
  term_TmVlv_PreCacPerc : Terminator
  term_Tm_AddWtrPmpFlgBusOff : Terminator
  term_Tm_AmbAirTp : Terminator
  term_Tm_CafDynRideFlg : Terminator
  term_Tm_CooltSwtVlvAuxHeatgOpenReq : Terminator
  term_Tm_EcuRunOnModReqRawFlg : Terminator
  term_Tm_ExhTp : Terminator
  term_Tm_FlgFanMotIndcnLampOnSubReq : Terminator
  term_Tm_FlgLoLvlTpCoolgIndcnLampOnReq : Terminator
  term_Tm_LtCcrTpDcDcSp : Terminator
  term_Tm_LtCcrTpEmInvSp : Terminator
  term_Tm_ProdModAcvFlg : Terminator
  term_ZFC_FlgColdChmb : Terminator
  term_ebg_rp_r : Terminator
  term_flg_ExhHeatgForFanLoaIncAcv : Terminator
  term_flg_MesCameoInca : Terminator
  term_flg_TmHtCcrVlvAgrReq : Terminator
  term_flg_TmHtCcrVlvAgrReqRels : Terminator
  term_flg_TmLtCcrEwpIcoReq : Terminator
  term_flg_TmLtCcrVlvReq : Terminator
  term_flg_TmLtCcrVlvReqEwpRo : Terminator
  term_flg_TmLtCcrVlvReqRels : Terminator
  term_flg_TmPumpRunOnReq : Terminator
  term_flg_TmPumpRunOnReqRels : Terminator
  term_flg_TmRelsDrvpPwrLimActd : Terminator
  term_flg_TmTpTcmProtnThCtl : Terminator
  term_fmiv08_r : Terminator
  term_nist_1uf_r : Terminator
  term_nst08 : Terminator
  term_perc_TmLtCcrEwpIcoReq : Terminator
  term_pw12r_r : Terminator
  term_sst_Baro_Res : Terminator
  term_sw_ped_r : Terminator
  term_tlst08 : Terminator
  term_ut_Trigger_Cyl_Cntr : Terminator
  term_vcanv05_r : Terminator
  term_vcanv08_r : Terminator
  term_vcanv16_r : Terminator
  term_volt_TmFanLoGenr : Terminator
  varCod_Cod_DPF_Mode : Constant  Value=ECM.VarCod.Cod_DPF_Mode
  varCod_Cod_Eng_AMG_Mode : Constant  Value=ECM.VarCod.Cod_Eng_AMG_Mode
  varCod_Cod_Eng_Diesel_Mode : Constant  Value=ECM.VarCod.Cod_Eng_Diesel_Mode
  varCod_Cod_Func_BoilProt : Constant  Value=ECM.VarCod.Cod_Func_BoilProt
  varCod_Cod_HDC_State : Constant  Value=ECM.VarCod.Cod_HDC_State
  varCod_Cod_HPP_Mode : Constant  Value=ECM.VarCod.Cod_HPP_Mode
  varCod_Cod_Model : Constant  Value=ECM.VarCod.Cod_Model
  varCod_Cod_SCR_Mode : Constant  Value=ECM.VarCod.Cod_SCR_Mode
  varCod_Cod_TM_CAS_Mode : Constant  Value=ECM.VarCod.Cod_TM_CAS_Mode
  varCod_Cod_TM_FC : Constant  Value=ECM.VarCod.Cod_TM_FC
  varCod_Cod_TM_HtrVlv_Mode : Constant  Value=ECM.VarCod.Cod_TM_HtrVlv_Mode
  varCod_Cod_TM_IAT_Mode : Constant  Value=ECM.VarCod.Cod_TM_IAT_Mode
  varCod_Cod_TM_Temp_NomVal_Mode : Constant  Value=ECM.VarCod.Cod_TM_Temp_NomVal_Mode
  varCod_Codn_FlgClpmp : Constant  Value=ECM.VarCod.Codn_FlgClpmp
  varCod_flg_CodnGb9 : Constant  Value=ECM.VarCod.flg_CodnGb9
  varCod_flg_CodnTmEngOilAirCool : Constant  Value=ECM.VarCod.flg_CodnTmEngOilAirCool
  varCod_flg_CodnTmEngRunngAftCoolgAcv : Constant  Value=ECM.VarCod.flg_CodnTmEngRunngAftCoolgAcv
  COMP_RunOn_Mode_Req : Outport
  CoolFan_Pwr_Req_Base : Outport  Port=2
  ECC_RotVlv_Posn_Req : Outport  Port=3
  ECU_RunOn_Mode_Req : Outport  Port=4
  EcmTm_FlgEngCoolgSysFlt : Outport  Port=5
  Ecm_CurCns48V : Outport  Port=6
  ExtAir_Temp_Mod : Outport  Port=7
  ExtAir_Temp_Mod_Sq : Outport  Port=8
  OilPump_Req_PWM : Outport  Port=9
  Sen_Oil_Temp : Outport  Port=10
  TM_CCRGA_Req : Outport  Port=11
  TM_CoolFan_StartCorrection : Outport  Port=12
  TM_ECT_Ref : Outport  Port=13
  TM_RegenWCRFan_Mode : Outport  Port=14
  TM_TROil_Shuttr_Req : Outport  Port=15
  TmHi_FlgQhtMemDmdOpgShttr : Outport  Port=16
  TmMdl_StandHeatIntglFac : Outport  Port=17
  TmPmp_EngClpmpLinReqPwm : Outport  Port=18
  TmPmp_EngClpmpPostRunModAcvFlg : Outport  Port=19
  TmPmp_THeatrPmpAftRunReq3 : Outport  Port=20
  Tm_LtCcrTpChAirSp : Outport  Port=21
  Tm_LtCcrTpSpRgnAct : Outport  Port=22
  flg_TestDiagCoolFanLinMod : Outport  Port=23
  perc_TestDiagCoolFanLinReq : Outport  Port=24
  wires:
  AdapAltitudeTempCorr_Coef/1 -> [L1]  "AdapAltitudeTempCorr_Coef"
  [L1] -> sfunction/30
  Eng_RelLoad/1 -> [L2]  "Eng_RelLoad"
  [L2] -> sfunction/31
  Eng_Spd/1 -> [L3]  "Eng_Spd"
  [L3] -> sfunction/32
  Veh_Spd/1 -> [L4]  "Veh_Spd"
  [L4] -> sfunction/33
  Ign_Mode/1 -> [L5]  "Ign_Mode"
  [L5] -> sfunction/34
  const_Emmo_PwrRecupForEbstrAvl/1 -> [L6]  "Emmo_PwrRecupForEbstrAvl"
  [L6] -> sfunction/35
  const_Emmo_PwrRecupForEbstrAvlSq/1 -> [L7]  "Emmo_PwrRecupForEbstrAvlSq"
  [L7] -> sfunction/36
  Emmo_VoltLinkPN48/1 -> [L8]  "Emmo_VoltLinkPN48"
  [L8] -> sfunction/37
  const_Emmo_VoltLinkPN48Sq/1 -> [L9]  "Emmo_VoltLinkPN48Sq"
  [L9] -> sfunction/38
  Hepm_PwrMax48VEcm/1 -> [L10]  "Hepm_PwrMax48VEcm"
  [L10] -> sfunction/39
  const_Hepm_PwrMax48VEcmSq/1 -> [L11]  "Hepm_PwrMax48VEcmSq"
  [L11] -> sfunction/40
  const_LIN_CP_ECP4TransCurr/1 -> [L12]  "LIN_CP_ECP4TransCurr"
  [L12] -> sfunction/41
  const_LIN_CP_ECP4TransCurrSq/1 -> [L13]  "LIN_CP_ECP4TransCurrSq"
  [L13] -> sfunction/42
  Net_EBoost_CurrCons/1 -> [L14]  "Net_EBoost_CurrCons"
  [L14] -> sfunction/43
  const_Net_EBoost_CurrConsSq/1 -> [L15]  "Net_EBoost_CurrConsSq"
  [L15] -> sfunction/44
  Pnct48V_VoltMinThdShutDwnEcm/1 -> [L16]  "Pnct48V_VoltMinThdShutDwnEcm"
  [L16] -> sfunction/45
  const_Pnct48V_VoltMinThdShutDwnEcmSq/1 -> [L17]  "Pnct48V_VoltMinThdShutDwnEcmSq"
  [L17] -> sfunction/46
  varCod_Cod_Eng_AMG_Mode/1 -> [L18]  "Cod_Eng_AMG_Mode"
  [L18] -> sfunction/47
  varCod_Cod_Func_BoilProt/1 -> [L19]  "Cod_Func_BoilProt"
  [L19] -> sfunction/48
  varCod_Cod_HPP_Mode/1 -> [L20]  "Cod_HPP_Mode"
  [L20] -> sfunction/49
  varCod_Cod_Model/1 -> [L21]  "Cod_Model"
  [L21] -> sfunction/50
  Dlay_ECTOut/1 -> [L22]  "ECTOut"
  [L22] -> sfunction/51
  Eng_RelLoad_Req/1 -> [L23]  "Eng_RelLoad_Req"
  [L23] -> sfunction/52
  Eng_Run_Mode/1 -> [L24]  "Eng_Run_Mode"
  [L24] -> sfunction/53
  const_EngCoolThOutTp_Tp/1 -> [L25]  "EngCoolThOutTp_Tp"
  [L25] -> sfunction/54
  const_ErrErs_Mode/1 -> [L26]  "ErrErs_Mode"
  [L26] -> sfunction/55
  LIN_CP_ECP4TransActlSpd/1 -> [L27]  "LIN_CP_ECP4TransActlSpd"
  [L27] -> sfunction/56
  const_LIN_CP_ECP4TransActlSpdSq/1 -> [L28]  "LIN_CP_ECP4TransActlSpdSq"
  [L28] -> sfunction/57
  const_LIN_CP_ECP4TransDryRunErr_State/1 -> [L29]  "LIN_CP_ECP4TransDryRunErr_State"
  [L29] -> sfunction/58
  LIN_CP_ECP4TransVoltStat/1 -> [L30]  "LIN_CP_ECP4TransVoltStat"
  [L30] -> sfunction/59
  const_LIN_CP_ECP4TransVoltStatSq/1 -> [L31]  "LIN_CP_ECP4TransVoltStatSq"
  [L31] -> sfunction/60
  const_Prcs_DiagRstFlg/1 -> [L32]  "Prcs_DiagRstFlg"
  [L32] -> sfunction/61
  TrqSetIgn_Mode_Req/1 -> [L33]  "TrqSetIgn_Mode_Req"
  [L33] -> sfunction/62
  TrqSetRes_Mode_Req/1 -> [L34]  "TrqSetRes_Mode_Req"
  [L34] -> sfunction/63
  const_Veh_Spd_Err_Mode/1 -> [L35]  "Veh_Spd_Err_Mode"
  [L35] -> sfunction/64
  const_FirstStrt_Mode/1 -> [L36]  "FirstStrt_Mode"
  [L36] -> sfunction/65
  Dlay_FirstStrt_Mode_EE/1 -> [L37]  "FirstStrt_Mode_EE"
  [L37] -> sfunction/66
  const_flg_PremAirTmDirt/1 -> [L38]  "flg_PremAirTmDirt"
  [L38] -> sfunction/67
  Dlay_IgnSwRun_Mode/1 -> [L39]  "IgnSwRun_Mode"
  [L39] -> sfunction/68
  const_RotVlvMalf_Mode/1 -> [L40]  "RotVlvMalf_Mode"
  [L40] -> sfunction/69
  AC_HtrVlv_Front_Req/1 -> [L41]  "AC_HtrVlv_Front_Req"
  [L41] -> sfunction/70
  const_AC_HtrVlv_Front_ReqSq/1 -> [L42]  "AC_HtrVlv_Front_ReqSq"
  [L42] -> sfunction/71
  const_AirFilOutTp_Sq/1 -> [L43]  "AirFilOutTp_Sq"
  [L43] -> sfunction/72
  const_AmbAirTp_Sq/1 -> [L44]  "AmbAirTp_Sq"
  [L44] -> sfunction/73
  AmbAirTp_Tp/1 -> [L45]  "AmbAirTp_Tp"
  [L45] -> sfunction/74
  const_CacInTp_Sq/1 -> [L46]  "CacInTp_Sq"
  [L46] -> sfunction/75
  CacInTp_Tp/1 -> [L47]  "CacInTp_Tp"
  [L47] -> sfunction/76
  const_Diag_DsblCntr_Resp/1 -> [L48]  "Diag_DsblCntr_Resp"
  [L48] -> sfunction/77
  const_ECF_Pwr_Req/1 -> [L49]  "ECF_Pwr_Req"
  [L49] -> sfunction/78
  Ecu_St/1 -> [L50]  "Ecu_St"
  [L50] -> sfunction/79
  const_EngCoolTp_Sq/1 -> [L51]  "EngCoolTp_Sq"
  [L51] -> sfunction/80
  EngCoolTp_Tp/1 -> [L52]  "EngCoolTp_Tp"
  [L52] -> sfunction/81
  const_EngOilTp_Sq/1 -> [L53]  "EngOilTp_Sq"
  [L53] -> sfunction/82
  EngOilTp_Tp/1 -> [L54]  "EngOilTp_Tp"
  [L54] -> sfunction/83
  Dlay_Exh_Temp/1 -> [L55]  "Exh_Temp"
  [L55] -> sfunction/84
  Dlay_flg_ChrgrAirCcrAcv/1 -> [L56]  "flg_ChrgrAirCcrAcv"
  [L56] -> sfunction/85
  IgnSwStrtr_Mode/1 -> [L57]  "IgnSwStrtr_Mode"
  [L57] -> sfunction/86
  Dlay_Shuttr_Pos_Req_I/1 -> [L58]  "Shuttr_Pos_Req_I"
  [L58] -> sfunction/87
  Dlay_TmFan_MalfFlg/1 -> [L59]  "TmFan_MalfFlg"
  [L59] -> sfunction/88
  const_TmFan_MalfFlgSq/1 -> [L60]  "TmFan_MalfFlgSq"
  [L60] -> sfunction/89
  Dlay_TM_ShttrDeIcing_ECTRef_I/1 -> [L61]  "TM_ShttrDeIcing_ECTRef_I"
  [L61] -> sfunction/90
  tp_ExhAtExhMnfld/1 -> [L62]  "tp_ExhAtExhMnfld"
  [L62] -> sfunction/91
  TrbInTp_Tp/1 -> [L63]  "TrbInTp_Tp"
  [L63] -> sfunction/92
  Bat_Volt/1 -> [L64]  "Bat_Volt"
  [L64] -> sfunction/93
  varCod_Codn_FlgClpmp/1 -> [L65]  "Codn_FlgClpmp"
  [L65] -> sfunction/94
  varCod_Cod_Eng_Diesel_Mode/1 -> [L66]  "Cod_Eng_Diesel_Mode"
  [L66] -> sfunction/95
  varCod_Cod_SCR_Mode/1 -> [L67]  "Cod_SCR_Mode"
  [L67] -> sfunction/96
  varCod_Cod_TM_IAT_Mode/1 -> [L68]  "Cod_TM_IAT_Mode"
  [L68] -> sfunction/97
  Dlay_EngShutOff_Time/1 -> [L69]  "EngShutOff_Time"
  [L69] -> sfunction/98
  Eng_Fuel_Mass_Flow_Calc/1 -> [L70]  "Eng_Fuel_Mass_Flow_Calc"
  [L70] -> sfunction/99
  const_Err_EngShutOff_Time/1 -> [L71]  "Err_EngShutOff_Time"
  [L71] -> sfunction/100
  MAF/1 -> [L72]  "MAF"
  [L72] -> sfunction/101
  ScrcmDos_THeatrPmpAftRunReq/1 -> [L73]  "ScrcmDos_THeatrPmpAftRunReq"
  [L73] -> sfunction/102
  TCM_Oil_Temp/1 -> [L74]  "TCM_Oil_Temp"
  [L74] -> sfunction/103
  const_TCM_Oil_TempSq/1 -> [L75]  "TCM_Oil_TempSq"
  [L75] -> sfunction/104
  const_TM_RegenActive_Mode/1 -> [L76]  "TM_RegenActive_Mode"
  [L76] -> sfunction/105
  Trans_OilTempHigh_Mode/1 -> [L77]  "Trans_OilTempHigh_Mode"
  [L77] -> sfunction/106
  const_ACCompr_RunMode_Plaus/1 -> [L78]  "ACCompr_RunMode_Plaus"
  [L78] -> sfunction/107
  APP/1 -> [L79]  "APP"
  [L79] -> sfunction/108
  varCod_Cod_DPF_Mode/1 -> [L80]  "Cod_DPF_Mode"
  [L80] -> sfunction/109
  varCod_Cod_HDC_State/1 -> [L81]  "Cod_HDC_State"
  [L81] -> sfunction/110
  const_Com_HPP_DrvProg/1 -> [L82]  "Com_HPP_DrvProg"
  [L82] -> sfunction/111
  const_DrProgram/1 -> [L83]  "DrProgram"
  [L83] -> sfunction/112
  ECU_Temp/1 -> [L84]  "ECU_Temp"
  [L84] -> sfunction/113
  EM2_InvrtTemp/1 -> [L85]  "EM2_InvrtTemp"
  [L85] -> sfunction/114
  const_EM2_InvrtTempSq/1 -> [L86]  "EM2_InvrtTempSq"
  [L86] -> sfunction/115
  Eng_Trq_Ind/1 -> [L87]  "Eng_Trq_Ind"
  [L87] -> sfunction/116
  Fuel_Temp/1 -> [L88]  "Fuel_Temp"
  [L88] -> sfunction/117
  Idle_Mode_Req/1 -> [L89]  "Idle_Mode_Req"
  [L89] -> sfunction/118
  IntkAir_Temp/1 -> [L90]  "IntkAir_Temp"
  [L90] -> sfunction/119
  const_Pn14Bat_Typ/1 -> [L91]  "Pn14Bat_Typ"
  [L91] -> sfunction/120
  const_TmMdl_TpTchQhtCor/1 -> [L92]  "TmMdl_TpTchQhtCor"
  [L92] -> sfunction/121
  const_TmPredCtl_EcTpSp/1 -> [L93]  "TmPredCtl_EcTpSp"
  [L93] -> sfunction/122
  const_Trlr_State/1 -> [L94]  "Trlr_State"
  [L94] -> sfunction/123
  VehMass_Wght_Pred/1 -> [L95]  "VehMass_Wght_Pred"
  [L95] -> sfunction/124
  const_WiprOutOfParkPosn/1 -> [L96]  "WiprOutOfParkPosn"
  [L96] -> sfunction/125
  AGC_ASSStop_Mode/1 -> [L97]  "AGC_ASSStop_Mode"
  [L97] -> sfunction/126
  AGKInit_Mode/1 -> [L98]  "AGKInit_Mode"
  [L98] -> sfunction/127
  varCod_Cod_TM_CAS_Mode/1 -> [L99]  "Cod_TM_CAS_Mode"
  [L99] -> sfunction/128
  varCod_Cod_TM_FC/1 -> [L100]  "Cod_TM_FC"
  [L100] -> sfunction/129
  const_Crash_Mode/1 -> [L101]  "Crash_Mode"
  [L101] -> sfunction/130
  const_DTM_Mode/1 -> [L102]  "DTM_Mode"
  [L102] -> sfunction/131
  const_EngHood_Plaus_Mode/1 -> [L103]  "EngHood_Plaus_Mode"
  [L103] -> sfunction/132
  const_Err_ECU_Temp_Mode/1 -> [L104]  "Err_ECU_Temp_Mode"
  [L104] -> sfunction/133
  Dlay_flg_PAFGCoolFanLinMod/1 -> [L105]  "flg_PAFGCoolFanLinMod"
  [L105] -> sfunction/134
  Gear_State/1 -> [L106]  "Gear_State"
  [L106] -> sfunction/135
  HDC_HybAggr_State/1 -> [L107]  "HDC_HybAggr_State"
  [L107] -> sfunction/136
  Dlay_LIN_CF_Spd_Req/1 -> [L108]  "LIN_CF_Spd_Req"
  [L108] -> sfunction/137
  Dlay_perc_PAFGCoolFanLinReq/1 -> [L109]  "perc_PAFGCoolFanLinReq"
  [L109] -> sfunction/138
  Eng_Trq/1 -> [L110]  "Eng_Trq"
  [L110] -> sfunction/139
  const_flg_PremAirGrdtFai/1 -> [L111]  "flg_PremAirGrdtFai"
  [L111] -> sfunction/140
  const_flg_PremAirPosFrameAcv/1 -> [L112]  "flg_PremAirPosFrameAcv"
  [L112] -> sfunction/141
  varCod_Cod_TM_HtrVlv_Mode/1 -> [L113]  "Cod_TM_HtrVlv_Mode"
  [L113] -> sfunction/142
  DFI_OprState/1 -> [L114]  "DFI_OprState"
  [L114] -> sfunction/143
  Err_ECT_low/1 -> [L115]  "Err_ECT_low"
  [L115] -> sfunction/144
  varCod_flg_CodnTmEngRunngAftCoolgAcv/1 -> [L116]  "flg_CodnTmEngRunngAftCoolgAcv"
  [L116] -> sfunction/145
  const_flg_TestDiagTmLtCcrVlvIcoMod/1 -> [L117]  "flg_TestDiagTmLtCcrVlvIcoMod"
  [L117] -> sfunction/146
  const_flg_TestDiagTmLtCcrVlvIcoReq/1 -> [L118]  "flg_TestDiagTmLtCcrVlvIcoReq"
  [L118] -> sfunction/147
  const_flg_TmHwCptSwtlEnag/1 -> [L119]  "flg_TmHwCptSwtlEnag"
  [L119] -> sfunction/148
  Dlay_TmHiTp_ThOpenSts/1 -> [L120]  "TmHiTp_ThOpenSts"
  [L120] -> sfunction/149
  const_TmTh_AcvThDiagOpgFlg/1 -> [L121]  "TmTh_AcvThDiagOpgFlg"
  [L121] -> sfunction/150
  Dlay_TM_Shttr_TjaErrIrrv_LIN/1 -> [L122]  "TM_Shttr_TjaErrIrrv_LIN"
  [L122] -> sfunction/151
  const_TM_Shttr_TjaErrIrrv_LINSq/1 -> [L123]  "TM_Shttr_TjaErrIrrv_LINSq"
  [L123] -> sfunction/152
  EM2_Cool_Req/1 -> [L124]  "EM2_Cool_Req"
  [L124] -> sfunction/153
  const_EM2_Cool_ReqSq/1 -> [L125]  "EM2_Cool_ReqSq"
  [L125] -> sfunction/154
  AGC_DTREngCutOff_Mode/1 -> [L126]  "AGC_DTREngCutOff_Mode"
  [L126] -> sfunction/155
  const_Bms48_StCntctrD/1 -> [L127]  "Bms48_StCntctrD"
  [L127] -> sfunction/156
  const_DiagcTstr_EngClpmpActFlg/1 -> [L128]  "DiagcTstr_EngClpmpActFlg"
  [L128] -> sfunction/157
  const_DiagcTstr_EngClpmpReqPwm/1 -> [L129]  "DiagcTstr_EngClpmpReqPwm"
  [L129] -> sfunction/158
  EngClpmp_FlgOnReq/1 -> [L130]  "EngClpmp_FlgOnReq"
  [L130] -> sfunction/159
  const_EngClpmp_FlgOnReqSq/1 -> [L131]  "EngClpmp_FlgOnReqSq"
  [L131] -> sfunction/160
  EngClpmp_PercPwrReq/1 -> [L132]  "EngClpmp_PercPwrReq"
  [L132] -> sfunction/161
  const_EngClpmp_PercPwrReqSq/1 -> [L133]  "EngClpmp_PercPwrReqSq"
  [L133] -> sfunction/162
  Hvac_StDefrstAcv/1 -> [L134]  "Hvac_StDefrstAcv"
  [L134] -> sfunction/163
  const_Hvac_StDefrstAcvSq/1 -> [L135]  "Hvac_StDefrstAcvSq"
  [L135] -> sfunction/164
  Dlay_TmClpmp_LtCcrGbRsgTpQvolReq/1 -> [L136]  "TmClpmp_LtCcrGbRsgTpQvolReq"
  [L136] -> sfunction/165
  const_TmClpmp_LtCcrGbRsgTpQvolReqSq/1 -> [L137]  "TmClpmp_LtCcrGbRsgTpQvolReqSq"
  [L137] -> sfunction/166
  const_TmClpmp_ThDiagClpmpPWM/1 -> [L138]  "TmClpmp_ThDiagClpmpPWM"
  [L138] -> sfunction/167
  const_LIN_CP_ECP4StEltlErr/1 -> [L139]  "LIN_CP_ECP4StEltlErr"
  [L139] -> sfunction/168
  const_LIN_CP_ECP4TransBlkErr_State/1 -> [L140]  "LIN_CP_ECP4TransBlkErr_State"
  [L140] -> sfunction/169
  const_LIN_CP_ECP4TransMon_StateSq/1 -> [L141]  "LIN_CP_ECP4TransMon_StateSq"
  [L141] -> sfunction/170
  const_LIN_CP_ECP4TransOvrCurrErr_St/1 -> [L142]  "LIN_CP_ECP4TransOvrCurrErr_St"
  [L142] -> sfunction/171
  const_LIN_CP_ECP4TransOvrTpErr_State/1 -> [L143]  "LIN_CP_ECP4TransOvrTpErr_State"
  [L143] -> sfunction/172
  const_LIN_CP_ECP4TransPostRun_StateSq/1 -> [L144]  "LIN_CP_ECP4TransPostRun_StateSq"
  [L144] -> sfunction/173
  const_LIN_CP_ECP4TransPwmIn_StateSq/1 -> [L145]  "LIN_CP_ECP4TransPwmIn_StateSq"
  [L145] -> sfunction/174
  const_LIN_CP_ECP4TransRpmRedStat/1 -> [L146]  "LIN_CP_ECP4TransRpmRedStat"
  [L146] -> sfunction/175
  const_LIN_CP_ECP4TransTgtSpdSq/1 -> [L147]  "LIN_CP_ECP4TransTgtSpdSq"
  [L147] -> sfunction/176
  const_LIN_CP_ECP4TransTpSq/1 -> [L148]  "LIN_CP_ECP4TransTpSq"
  [L148] -> sfunction/177
  const_LIN_CP_ECP4TransVoltErr_State/1 -> [L149]  "LIN_CP_ECP4TransVoltErr_State"
  [L149] -> sfunction/178
  const_ThrInTp_Sq/1 -> [L150]  "ThrInTp_Sq"
  [L150] -> sfunction/179
  ag_CamsftExhSp/1 -> [L151]  "ag_CamsftExhSp"
  [L151] -> sfunction/180
  ag_CamsftIntkSp/1 -> [L152]  "ag_CamsftIntkSp"
  [L152] -> sfunction/181
  AmbAirP_P/1 -> [L153]  "AmbAirP_P"
  [L153] -> sfunction/182
  const_AmbAirP_Sq/1 -> [L154]  "AmbAirP_Sq"
  [L154] -> sfunction/183
  DFSO_Mode/1 -> [L155]  "DFSO_Mode"
  [L155] -> sfunction/184
  const_DiagcTstr_PcdOilPDeacvnKmFlg/1 -> [L156]  "DiagcTstr_PcdOilPDeacvnKmFlg"
  [L156] -> sfunction/185
  Dspl_EngShutOff_Time/1 -> [L157]  "Dspl_EngShutOff_Time"
  [L157] -> sfunction/186
  Eng_Actl_OpMode/1 -> [L158]  "Eng_Actl_OpMode"
  [L158] -> sfunction/187
  Eng_State_Actl/1 -> [L159]  "Eng_State_Actl"
  [L159] -> sfunction/188
  EngOilP_P/1 -> [L160]  "EngOilP_P"
  [L160] -> sfunction/189
  const_EngOilP_Sq/1 -> [L161]  "EngOilP_Sq"
  [L161] -> sfunction/190
  Odo_Abs_Long/1 -> [L162]  "Odo_Abs_Long"
  [L162] -> sfunction/191
  Dlay_Tm_FlgEngOilHiPReq/1 -> [L163]  "Tm_FlgEngOilHiPReq"
  [L163] -> sfunction/192
  ECT/1 -> [L164]  "ECT"
  [L164] -> sfunction/193
  FRT_Sens/1 -> [L165]  "FRT_Sens"
  [L165] -> sfunction/194
  Fu_Mp1/1 -> [L166]  "Fu_Mp1"
  [L166] -> sfunction/195
  Injr_Tp/1 -> [L167]  "Injr_Tp"
  [L167] -> sfunction/196
  n_Eng/1 -> [L168]  "n_Eng"
  [L168] -> sfunction/197
  const_Exh_Temp_Err_Mode/1 -> [L169]  "Exh_Temp_Err_Mode"
  [L169] -> sfunction/198
  AAP/1 -> [L170]  "AAP"
  [L170] -> sfunction/199
  const_EOM_Actl_OpMode/1 -> [L171]  "EOM_Actl_OpMode"
  [L171] -> sfunction/200
  varCod_Cod_TM_Temp_NomVal_Mode/1 -> [L172]  "Cod_TM_Temp_NomVal_Mode"
  [L172] -> sfunction/201
  const_Err_MAF_Mode/1 -> [L173]  "Err_MAF_Mode"
  [L173] -> sfunction/202
  const_flg_PremAirTmDirtT/1 -> [L174]  "flg_PremAirTmDirtT"
  [L174] -> sfunction/203
  const_Hpmc_StPlgnOpmdReq/1 -> [L175]  "Hpmc_StPlgnOpmdReq"
  [L175] -> sfunction/204
  AT2_Mode/1 -> [L176]  "AT2_Mode"
  [L176] -> sfunction/205
  ExtAir_Temp_Raw/1 -> [L177]  "ExtAir_Temp_Raw"
  [L177] -> sfunction/206
  varCod_flg_CodnGb9/1 -> [L178]  "flg_CodnGb9"
  [L178] -> sfunction/207
  const_flg_PremAirTmOpen/1 -> [L179]  "flg_PremAirTmOpen"
  [L179] -> sfunction/208
  IC_Knk_Red_Avg/1 -> [L180]  "IC_Knk_Red_Avg"
  [L180] -> sfunction/209
  IC_Knk_Red_Avg_Actv/1 -> [L181]  "IC_Knk_Red_Avg_Actv"
  [L181] -> sfunction/210
  const_Trlr_StateSq/1 -> [L182]  "Trlr_StateSq"
  [L182] -> sfunction/211
  AirFilOutTp_Tp/1 -> [L183]  "AirFilOutTp_Tp"
  [L183] -> sfunction/212
  EngCoolTp_TpMdl/1 -> [L184]  "EngCoolTp_TpMdl"
  [L184] -> sfunction/213
  IMAT/1 -> [L185]  "IMAT"
  [L185] -> sfunction/214
  const_CarHtr_EngStrt_Mode/1 -> [L186]  "CarHtr_EngStrt_Mode"
  [L186] -> sfunction/215
  Eng_Cyc_Time/1 -> [L187]  "Eng_Cyc_Time"
  [L187] -> sfunction/216
  varCod_flg_CodnTmEngOilAirCool/1 -> [L188]  "flg_CodnTmEngOilAirCool"
  [L188] -> sfunction/217
  K15/1 -> [L189]  "K15"
  [L189] -> sfunction/1
  const_timePostdrive/1 -> [L190]  "timePostdrive"
  [L190] -> sfunction/2
  eeprom_TM_CCRGAEATHi/1 -> [L191]  "TM_CCRGAEATHi"
  [L191] -> sfunction/3
  eeprom_TM_CCRGAEATLo/1 -> [L192]  "TM_CCRGAEATLo"
  [L192] -> sfunction/4
  eeprom_TM_CCRGAEATMid/1 -> [L193]  "TM_CCRGAEATMid"
  [L193] -> sfunction/5
  eeprom_TM_CCRGA_Hi/1 -> [L194]  "TM_CCRGA_Hi"
  [L194] -> sfunction/6
  eeprom_TM_CCRGA_Lo/1 -> [L195]  "TM_CCRGA_Lo"
  [L195] -> sfunction/7
  eeprom_TM_CCRGA_Mid/1 -> [L196]  "TM_CCRGA_Mid"
  [L196] -> sfunction/8
  eeprom_TM_CCRGA_act/1 -> [L197]  "TM_CCRGA_act"
  [L197] -> sfunction/9
  eeprom_TM_ECT_Ref_Cntr_HT/1 -> [L198]  "TM_ECT_Ref_Cntr_HT"
  [L198] -> sfunction/10
  eeprom_TM_ECT_Ref_Cntr_LT/1 -> [L199]  "TM_ECT_Ref_Cntr_LT"
  [L199] -> sfunction/11
  eeprom_TM_LTCoolPump_RunTime6/1 -> [L200]  "TM_LTCoolPump_RunTime6"
  [L200] -> sfunction/12
  eeprom_TOil_ShutOff/1 -> [L201]  "TOil_ShutOff"
  [L201] -> sfunction/13
  eeprom_TmEcTpSp_CtrEcuTp0/1 -> [L202]  "TmEcTpSp_CtrEcuTp0"
  [L202] -> sfunction/14
  eeprom_TmEcTpSp_CtrEcuTp1/1 -> [L203]  "TmEcTpSp_CtrEcuTp1"
  [L203] -> sfunction/15
  eeprom_TmEcTpSp_CtrEcuTp2/1 -> [L204]  "TmEcTpSp_CtrEcuTp2"
  [L204] -> sfunction/16
  eeprom_TmEcTpSp_CtrEcuTp3/1 -> [L205]  "TmEcTpSp_CtrEcuTp3"
  [L205] -> sfunction/17
  eeprom_TmEcTpSp_CtrEcuTp4/1 -> [L206]  "TmEcTpSp_CtrEcuTp4"
  [L206] -> sfunction/18
  eeprom_TmEcTpSp_CtrEcuTp5/1 -> [L207]  "TmEcTpSp_CtrEcuTp5"
  [L207] -> sfunction/19
  eeprom_TmEcTpSp_CtrEcuTp6/1 -> [L208]  "TmEcTpSp_CtrEcuTp6"
  [L208] -> sfunction/20
  eeprom_TmEcTpSp_CtrEcuTp7/1 -> [L209]  "TmEcTpSp_CtrEcuTp7"
  [L209] -> sfunction/21
  eeprom_TmEcTpSp_CtrEcuTp8/1 -> [L210]  "TmEcTpSp_CtrEcuTp8"
  [L210] -> sfunction/22
  eeprom_TmEcTpSp_CtrEcuTp9/1 -> [L211]  "TmEcTpSp_CtrEcuTp9"
  [L211] -> sfunction/23
  eeprom_TmEcTpSp_TpEcuCtrDiRam/1 -> [L212]  "TmEcTpSp_TpEcuCtrDiRam"
  [L212] -> sfunction/24
  eeprom_TmHi_FacTCor2Ee/1 -> [L213]  "TmHi_FacTCor2Ee"
  [L213] -> sfunction/25
  eeprom_TmPcdLrng_CtlrFctCoefY100/1 -> [L214]  "TmPcdLrng_CtlrFctCoefY100"
  [L214] -> sfunction/26
  eeprom_TmPcdLrng_CtlrFctCoefY20/1 -> [L215]  "TmPcdLrng_CtlrFctCoefY20"
  [L215] -> sfunction/27
  eeprom_TmPcd_EepromPDeacvnOdoS/1 -> [L216]  "TmPcd_EepromPDeacvnOdoS"
  [L216] -> sfunction/28
  eeprom_TmPmp_TpQhtTchDram/1 -> [L217]  "TmPmp_TpQhtTchDram"
  [L217] -> sfunction/29
  const_modIn_Trigger_Cyl_Cntr/1 -> [L218]  "modIn_Trigger_Cyl_Cntr"
  [L218] -> sfunction/218
  [L221] -> term_AC_HtrVlv_Front_Plaus_Req/1
  sfunction/1 -> [L221]
  [L222] -> term_AC_HtrVlv_Front_Plaus_ReqSq/1
  sfunction/2 -> [L222]
  [L223] -> term_DiagcTstr_EngClpmpActSpd/1
  sfunction/3 -> [L223]
  [L224] -> term_Diagc_FlgNEngMinMaxReq12/1
  sfunction/4 -> [L224]
  [L225] -> term_Diagc_NEngMinMaxReq12/1
  sfunction/5 -> [L225]
  [L226] -> term_Diagc_StPrioReq12/1
  sfunction/6 -> [L226]
  [L227] -> term_Diagc_StWpReq12/1
  sfunction/7 -> [L227]
  [L228] -> term_Diagc_TqMaxReq12/1
  sfunction/8 -> [L228]
  [L229] -> term_Diagc_TqMinReq12/1
  sfunction/9 -> [L229]
  [L230] -> term_Diagc_TqOptmReq12/1
  sfunction/10 -> [L230]
  [L231] -> term_ECF_PwrReq_Plaus/1
  sfunction/11 -> [L231]
  [L232] -> term_ECTOut_Raw/1
  sfunction/12 -> [L232]
  [L233] -> term_Err_ECTOut_Mode/1
  sfunction/13 -> [L233]
  [L234] -> term_Err_IntkAir_Temp_Mode/1
  sfunction/14 -> [L234]
  [L235] -> ExtAir_Temp_Mod/1
  sfunction/15 -> [L235]
  [L236] -> term_ExtAir_Temp_Mod_SNA_Mode/1
  sfunction/16 -> [L236]
  [L237] -> ExtAir_Temp_Mod_Sq/1
  sfunction/17 -> [L237]
  [L238] -> term_FanMalf_Mode/1
  sfunction/18 -> [L238]
  [L239] -> term_FanMalf_Mode_LIN/1
  sfunction/19 -> [L239]
  [L240] -> term_FanMalf_Mode_LINSq/1
  sfunction/20 -> [L240]
  [L241] -> term_flg_TmLtCcrEwpIcoReq/1
  sfunction/21 -> [L241]
  [L242] -> term_OilPump_SwitchState/1
  sfunction/22 -> [L242]
  [L243] -> term_Sen_Oil_Temp2/1
  sfunction/23 -> [L243]
  [L244] -> term_Sen_Oil_Temp2_SNA_Mode/1
  sfunction/24 -> [L244]
  [L245] -> term_Shuttr_Pos_Mode/1
  sfunction/25 -> [L245]
  [L246] -> term_Shuttr_Pos_Req/1
  sfunction/26 -> [L246]
  [L247] -> term_TmLtCcr_CacTp/1
  sfunction/27 -> [L247]
  [L248] -> term_TmLtCcr_CacTpSq/1
  sfunction/28 -> [L248]
  [L249] -> term_TmPmp_EngClpmpLinReqPwmCoorr/1
  sfunction/29 -> [L249]
  [L250] -> term_TmSigIf_StEcu/1
  sfunction/30 -> [L250]
  [L251] -> term_Tm_AmbAirTp/1
  sfunction/31 -> [L251]
  [L252] -> term_TM_CP_Req_PWM/1
  sfunction/32 -> [L252]
  [L253] -> term_Tm_ExhTp/1
  sfunction/33 -> [L253]
  [L254] -> term_TM_idxTmInCpc/1
  sfunction/34 -> [L254]
  [L255] -> term_TM_IgnSwStrtr_Mode/1
  sfunction/35 -> [L255]
  [L256] -> term_Tm_ProdModAcvFlg/1
  sfunction/36 -> [L256]
  [L257] -> term_TM_ShttrDeIcing_ECTRef/1
  sfunction/37 -> [L257]
  [L258] -> term_ErrEntry_EltFanMalfErr/1
  sfunction/38 -> [L258]
  [L259] -> term_ErrEntry_EltShttrMalfErr/1
  sfunction/39 -> [L259]
  [L260] -> term_TmClpmpErr_ErrSig/1
  sfunction/40 -> [L260]
  [L261] -> term_TmClpmp_BlkErrSym/1
  sfunction/41 -> [L261]
  [L262] -> term_TmClpmp_DryRunErrSym/1
  sfunction/42 -> [L262]
  [L263] -> term_TmClpmp_Ecp4ComErrMsgLost/1
  sfunction/43 -> [L263]
  [L264] -> term_TmClpmp_ElPmpErrMod/1
  sfunction/44 -> [L264]
  [L265] -> term_TmClpmp_EltErrSym/1
  sfunction/45 -> [L265]
  [L266] -> term_TmClpmp_ErrModIrrvFlg/1
  sfunction/46 -> [L266]
  [L267] -> term_TmClpmp_OverCurErrSym/1
  sfunction/47 -> [L267]
  [L268] -> term_TmClpmp_ReqFltModFlg/1
  sfunction/48 -> [L268]
  [L269] -> term_TmClpmp_VoltErrSym/1
  sfunction/49 -> [L269]
  [L270] -> term_TmPmp_ClpmpHiNErrFlg/1
  sfunction/50 -> [L270]
  [L271] -> term_TmPmp_ClpmpLoNErrFlg/1
  sfunction/51 -> [L271]
  [L272] -> term_CoolFan_MAF_Req/1
  sfunction/52 -> [L272]
  [L273] -> term_flg_MesCameoInca/1
  sfunction/53 -> [L273]
  [L274] -> term_flg_TmRelsDrvpPwrLimActd/1
  sfunction/54 -> [L274]
  [L275] -> term_LRS_Mode/1
  sfunction/55 -> [L275]
  [L276] -> term_TM_CAF_CT_ECT_H/1
  sfunction/56 -> [L276]
  [L277] -> term_TM_CAF_CT_ECT_L/1
  sfunction/57 -> [L277]
  [L278] -> term_TM_CAF_CT_ECU_Temp_Req/1
  sfunction/58 -> [L278]
  [L279] -> term_TM_CAF_CT_Exh_Temp_Req2/1
  sfunction/59 -> [L279]
  [L280] -> term_TM_CAF_CT_FanLoadInc_Req/1
  sfunction/60 -> [L280]
  [L281] -> term_TM_CAF_CT_Fuel_Temp_Req/1
  sfunction/61 -> [L281]
  [L282] -> term_TM_CAF_CT_HI_Req/1
  sfunction/62 -> [L282]
  [L283] -> term_TM_CAF_Max_Req_Stop/1
  sfunction/63 -> [L283]
  [L284] -> term_Tm_CafDynRideFlg/1
  sfunction/64 -> [L284]
  [L285] -> term_TM_Eng_Pwr_Ind/1
  sfunction/65 -> [L285]
  [L286] -> term_TmFan_FlgCooltReq/1
  sfunction/66 -> [L286]
  [L287] -> term_TmFan_PrevnSmkFmtAftRunFlg/1
  sfunction/67 -> [L287]
  [L288] -> term_volt_TmFanLoGenr/1
  sfunction/68 -> [L288]
  [L289] -> term_ACComprOff_FanMalf/1
  sfunction/69 -> [L289]
  [L290] -> term_CoolFan_Pwr_Req/1
  sfunction/70 -> [L290]
  [L291] -> CoolFan_Pwr_Req_Base/1
  sfunction/71 -> [L291]
  [L292] -> term_OilTemp_Mode/1
  sfunction/72 -> [L292]
  [L293] -> term_TM_ASSStopMode_OffDly/1
  sfunction/73 -> [L293]
  [L294] -> term_TM_CAF_Cod_TM_FC_Bit0/1
  sfunction/74 -> [L294]
  [L295] -> term_TM_CAF_VL_elViscoFan_Mode/1
  sfunction/75 -> [L295]
  [L296] -> term_TM_CoolFanPwrReq_Lim/1
  sfunction/76 -> [L296]
  [L297] -> term_TM_Eng_Run_Mode/1
  sfunction/77 -> [L297]
  [L298] -> term_TM_Eng_Run_Mode_Stop/1
  sfunction/78 -> [L298]
  [L299] -> term_TmFan_DiagAcvFlg/1
  sfunction/79 -> [L299]
  [L300] -> term_Fu_TpInjrTip/1
  sfunction/80 -> [L300]
  [L301] -> term_TmClpmp_PmpCtlRawPwm/1
  sfunction/81 -> [L301]
  [L302] -> term_ErrEntry_Koch/1
  sfunction/82 -> [L302]
  [L303] -> term_RelLoad_OvrHtgPrvn/1
  sfunction/83 -> [L303]
  [L304] -> term_RelLoad_OvrHtgPrvn_Mode/1
  sfunction/84 -> [L304]
  [L305] -> term_TM_ECT_Ref_Mn_en/1
  sfunction/85 -> [L305]
  [L306] -> term_TM_ECT_Ref_Mn_Load/1
  sfunction/86 -> [L306]
  [L307] -> TM_ECT_Ref/1
  sfunction/87 -> [L307]
  [L308] -> term_AC_MAF_Req/1
  sfunction/88 -> [L308]
  [L309] -> term_ClpmpRsg_AftRunReqSt/1
  sfunction/89 -> [L309]
  [L310] -> term_ClpmpRsg_NReq/1
  sfunction/90 -> [L310]
  [L311] -> term_Cod_Func_SGStrat/1
  sfunction/91 -> [L311]
  [L312] -> term_Com_HPP_DrvProgSq/1
  sfunction/92 -> [L312]
  [L313] -> COMP_RunOn_Mode_Req/1
  sfunction/93 -> [L313]
  [L314] -> term_CoolFan_Pwr_Req_RunOn/1
  sfunction/94 -> [L314]
  [L315] -> term_CoolFan_Pwr_Req_RunOn_Ok/1
  sfunction/95 -> [L315]
  [L316] -> term_CoolPump_Mode_Req/1
  sfunction/96 -> [L316]
  [L317] -> term_CoolPump_TCM_Mode_Req/1
  sfunction/97 -> [L317]
  [L318] -> term_CrkcsEvapn_FlgDaiLimEvap/1
  sfunction/98 -> [L318]
  [L319] -> term_CylBank1_FIRate_Rel/1
  sfunction/99 -> [L319]
  [L320] -> term_CylBank2_FIRate_Rel/1
  sfunction/100 -> [L320]
  [L321] -> term_Dpf_FlgRgnReq/1
  sfunction/101 -> [L321]
  [L322] -> term_ECU_RunOn_CoolFan_Req/1
  sfunction/102 -> [L322]
  [L323] -> term_ECU_RunOn_LinShuttr_Req/1
  sfunction/103 -> [L323]
  [L324] -> term_EGR_VlvPos/1
  sfunction/104 -> [L324]
  [L325] -> term_EGR_VlvPos_Err_Mode/1
  sfunction/105 -> [L325]
  [L326] -> term_EgrVlv2Posn/1
  sfunction/106 -> [L326]
  [L327] -> term_Eng_PercIntFanReq/1
  sfunction/107 -> [L327]
  sfunction/108 -> [L329]
  sfunction/109 -> [L332]
  sfunction/110 -> [L335]
  sfunction/111 -> [L338]
  sfunction/112 -> [L341]
  [L343] -> term_EomRampCo_StEomActDes/1
  sfunction/113 -> [L343]
  [L344] -> term_Err_Eng_Spd_Mode/1
  sfunction/114 -> [L344]
  [L345] -> term_EtdRgn_TpLoCcrDmd/1
  sfunction/115 -> [L345]
  [L346] -> term_Exh_Air_FlowFlt/1
  sfunction/116 -> [L346]
  [L347] -> term_FIRate_Fuel/1
  sfunction/117 -> [L347]
  [L348] -> term_FIRate_Trq/1
  sfunction/118 -> [L348]
  [L349] -> term_flg_ExhHeatgForFanLoaIncAcv/1
  sfunction/119 -> [L349]
  [L350] -> flg_TestDiagCoolFanLinMod/1
  sfunction/120 -> [L350]
  [L351] -> term_FuTpMdl/1
  sfunction/121 -> [L351]
  [L352] -> term_HtrVlvMalf_Mode/1
  sfunction/122 -> [L352]
  [L353] -> term_Inj_VolCyl/1
  sfunction/123 -> [L353]
  [L354] -> term_IntkAir_Temp2/1
  sfunction/124 -> [L354]
  [L355] -> term_LIN_CP_ECP4TransVoltSq/1
  sfunction/125 -> [L355]
  [L356] -> term_LIN_CP_ECP4WakeupStatSq/1
  sfunction/126 -> [L356]
  [L357] -> term_LTVlv_Mode_Req/1
  sfunction/127 -> [L357]
  [L358] -> term_Net_Eboost_CoolMassFlow/1
  sfunction/128 -> [L358]
  [L359] -> term_O2S_Ctrl2_Mode/1
  sfunction/129 -> [L359]
  [L360] -> term_O2SnsrFac2/1
  sfunction/130 -> [L360]
  [L361] -> perc_TestDiagCoolFanLinReq/1
  sfunction/131 -> [L361]
  [L362] -> term_perc_TmLtCcrEwpIcoReq/1
  sfunction/132 -> [L362]
  [L363] -> term_RailDiag_EnaFlg/1
  sfunction/133 -> [L363]
  [L364] -> term_SCR_DPDV_tUDosVlvPstFlt1/1
  sfunction/134 -> [L364]
  [L365] -> term_SenDiagHdr2/1
  sfunction/135 -> [L365]
  [L366] -> term_SenDiagLamSon2Unplaus/1
  sfunction/136 -> [L366]
  [L367] -> term_SenDiagSensSigErr2/1
  sfunction/137 -> [L367]
  [L368] -> term_ShuttrMalf_Mode/1
  sfunction/138 -> [L368]
  [L369] -> term_Sppl_TpCmprOutMdl2/1
  sfunction/139 -> [L369]
  [L370] -> term_TM_CAF_TR_EnC2/1
  sfunction/140 -> [L370]
  [L371] -> term_TM_CAF_TR_TGET_Req/1
  sfunction/141 -> [L371]
  [L372] -> term_TM_CoolFan_RO_Mode_Req/1
  sfunction/142 -> [L372]
  [L373] -> term_TM_CoolFanPwrReq_elVisco/1
  sfunction/143 -> [L373]
  [L374] -> term_Tm_CooltSwtVlvAuxHeatgOpenReq/1
  sfunction/144 -> [L374]
  [L375] -> term_TM_CP_CTR_AC/1
  sfunction/145 -> [L375]
  [L376] -> term_TM_ECF_DPFPwrReq/1
  sfunction/146 -> [L376]
  [L377] -> term_TM_ECF_DPFPwrReqMan/1
  sfunction/147 -> [L377]
  [L378] -> term_TM_ECF_LTCrct_Req_ECC/1
  sfunction/148 -> [L378]
  [L379] -> term_TM_ECF_SFT_Req/1
  sfunction/149 -> [L379]
  [L380] -> term_Tm_FlgFanMotIndcnLampOnSubReq/1
  sfunction/150 -> [L380]
  [L381] -> term_Tm_FlgLoLvlTpCoolgIndcnLampOnReq/1
  sfunction/151 -> [L381]
  [L382] -> term_TM_LTCoolPump_RunTime6/1
  sfunction/152 -> [L382]
  [L383] -> term_TM_PC_Req/1
  sfunction/153 -> [L383]
  [L384] -> term_TM_PFltRegenDemand_Mode/1
  sfunction/154 -> [L384]
  [L385] -> TM_RegenWCRFan_Mode/1
  sfunction/155 -> [L385]
  [L386] -> term_TM_Shttr_TjaErrIrrv/1
  sfunction/156 -> [L386]
  [L387] -> term_TM_TROil_ECTRef/1
  sfunction/157 -> [L387]
  [L388] -> term_TM_TROil_ECTRefVlv/1
  sfunction/158 -> [L388]
  [L389] -> TM_TROil_Shuttr_Req/1
  sfunction/159 -> [L389]
  [L390] -> term_TmBms_EcuRunOnReqFlg/1
  sfunction/160 -> [L390]
  [L391] -> term_TmPmp_RsgCcrEcuRunOnReqFlg/1
  sfunction/161 -> [L391]
  [L392] -> term_TmPmpLtCcr_EcuRunOnReqFlg/1
  sfunction/162 -> [L392]
  [L393] -> term_TmRsvBms_EcuRunOnReqFlg/1
  sfunction/163 -> [L393]
  [L394] -> term_TmRsvLtCcr_EcuRunOnReqFlg/1
  sfunction/164 -> [L394]
  [L395] -> term_TmVlv_PreCacPerc/1
  sfunction/165 -> [L395]
  [L396] -> term_ZFC_FlgColdChmb/1
  sfunction/166 -> [L396]
  [L397] -> term_TM_CoolFan_RO_Mode/1
  sfunction/167 -> [L397]
  [L398] -> TM_CoolFan_StartCorrection/1
  sfunction/168 -> [L398]
  [L399] -> term_TM_ISRD_Req/1
  sfunction/169 -> [L399]
  [L400] -> term_TM_RO_curHL/1
  sfunction/170 -> [L400]
  [L401] -> term_TM_RO_TCorrection2/1
  sfunction/171 -> [L401]
  [L402] -> term_TM_StopDsabl_Mode/1
  sfunction/172 -> [L402]
  [L403] -> term_TmHi_FacTCor2EeRead/1
  sfunction/173 -> [L403]
  [L404] -> TmHi_FlgQhtMemDmdOpgShttr/1
  sfunction/174 -> [L404]
  [L405] -> TmMdl_StandHeatIntglFac/1
  sfunction/175 -> [L405]
  [L406] -> term_TmClpmp_ActlElVolt/1
  sfunction/176 -> [L406]
  [L407] -> term_TM_ECT_Ref_Mn_Freeze/1
  sfunction/177 -> [L407]
  [L408] -> term_ebg_rp_r/1
  sfunction/178 -> [L408]
  [L409] -> term_fmiv08_r/1
  sfunction/179 -> [L409]
  [L410] -> term_nist_1uf_r/1
  sfunction/180 -> [L410]
  [L411] -> term_nst08/1
  sfunction/181 -> [L411]
  [L412] -> term_pw12r_r/1
  sfunction/182 -> [L412]
  [L413] -> term_sst_Baro_Res/1
  sfunction/183 -> [L413]
  [L414] -> term_sw_ped_r/1
  sfunction/184 -> [L414]
  [L415] -> term_tlst08/1
  sfunction/185 -> [L415]
  [L416] -> term_vcanv05_r/1
  sfunction/186 -> [L416]
  [L417] -> term_vcanv08_r/1
  sfunction/187 -> [L417]
  [L418] -> term_vcanv16_r/1
  sfunction/188 -> [L418]
  [L419] -> term_TmReqMinPremAirDirtFlag/1
  sfunction/189 -> [L419]
  [L420] -> term_TM_ECT_Ref_Mx/1
  sfunction/190 -> [L420]
  [L421] -> term_TM_ECT_Ref_PremADiagOk/1
  sfunction/191 -> [L421]
  [L422] -> Tm_LtCcrTpChAirSp/1
  sfunction/192 -> [L422]
  [L423] -> term_Tm_LtCcrTpDcDcSp/1
  sfunction/193 -> [L423]
  [L424] -> term_Tm_LtCcrTpEmInvSp/1
  sfunction/194 -> [L424]
  [L425] -> Tm_LtCcrTpSpRgnAct/1
  sfunction/195 -> [L425]
  [L426] -> term_TM_AddWtrPmp_On_Req/1
  sfunction/196 -> [L426]
  [L427] -> term_Tm_AddWtrPmpFlgBusOff/1
  sfunction/197 -> [L427]
  [L428] -> term_TM_TrsmWtrPmp_On_Req/1
  sfunction/198 -> [L428]
  [L429] -> term_TmPmp_FlgChrgrEwpHeatrReq/1
  sfunction/199 -> [L429]
  [L430] -> term_TmPmp_THeatrPmpAftRunReq1/1
  sfunction/200 -> [L430]
  [L431] -> TmPmp_THeatrPmpAftRunReq3/1
  sfunction/201 -> [L431]
  [L432] -> term_TmPmp_THeatrPmpAftRunReq6/1
  sfunction/202 -> [L432]
  [L433] -> term_TmPmp_TpQhtTch/1
  sfunction/203 -> [L433]
  [L434] -> term_EcmTm_FlgEngCoolgSysErr/1
  sfunction/204 -> [L434]
  [L435] -> EcmTm_FlgEngCoolgSysFlt/1
  sfunction/205 -> [L435]
  [L436] -> term_NetCoorr_FlgEcmLin2AcvnReq/1
  sfunction/206 -> [L436]
  [L437] -> term_TmClpmp_EcuOnReqFlg/1
  sfunction/207 -> [L437]
  [L438] -> term_TmPmp_EngClpmpEMOoff/1
  sfunction/208 -> [L438]
  [L439] -> TmPmp_EngClpmpLinReqPwm/1
  sfunction/209 -> [L439]
  [L440] -> TmPmp_EngClpmpPostRunModAcvFlg/1
  sfunction/210 -> [L440]
  [L441] -> ECC_RotVlv_Posn_Req/1
  sfunction/211 -> [L441]
  [L442] -> term_flg_TmHtCcrVlvAgrReq/1
  sfunction/212 -> [L442]
  [L443] -> term_flg_TmHtCcrVlvAgrReqRels/1
  sfunction/213 -> [L443]
  [L444] -> term_flg_TmLtCcrVlvReq/1
  sfunction/214 -> [L444]
  [L445] -> term_flg_TmLtCcrVlvReqEwpRo/1
  sfunction/215 -> [L445]
  [L446] -> term_flg_TmLtCcrVlvReqRels/1
  sfunction/216 -> [L446]
  [L447] -> term_flg_TmPumpRunOnReq/1
  sfunction/217 -> [L447]
  [L448] -> term_flg_TmPumpRunOnReqRels/1
  sfunction/218 -> [L448]
  [L449] -> term_HtrVlv_Mode_Req/1
  sfunction/219 -> [L449]
  [L450] -> term_HtrVlv_State/1
  sfunction/220 -> [L450]
  [L451] -> term_TM_RotV_LimPos/1
  sfunction/221 -> [L451]
  [L452] -> term_TmHeatrVlv_EcuRunOnReqFlg/1
  sfunction/222 -> [L452]
  [L453] -> term_flg_TmTpTcmProtnThCtl/1
  sfunction/223 -> [L453]
  [L454] -> term_TM_CCRCT_HV_Open/1
  sfunction/224 -> [L454]
  [L455] -> term_TM_RotV_Ref/1
  sfunction/225 -> [L455]
  [L456] -> Sen_Oil_Temp/1
  sfunction/226 -> [L456]
  [L457] -> term_Sen_Oil_Temp_Init_Mode/1
  sfunction/227 -> [L457]
  [L458] -> term_Sen_Oil_Temp_SNA_Mode/1
  sfunction/228 -> [L458]
  [L459] -> term_Sen_Oil_Temp_Sq/1
  sfunction/229 -> [L459]
  [L460] -> term_TOil_Mdl_Int_Out/1
  sfunction/230 -> [L460]
  [L461] -> term_TOIL_Sensor_dis/1
  sfunction/231 -> [L461]
  [L462] -> term_TM_CCRCTExtAir_Temp/1
  sfunction/232 -> [L462]
  [L463] -> term_TM_CCRGAStep/1
  sfunction/233 -> [L463]
  [L464] -> term_TM_CCRGA_Hi_out/1
  sfunction/234 -> [L464]
  [L465] -> term_TM_CCRGA_Lo_out/1
  sfunction/235 -> [L465]
  [L466] -> term_TM_CCRGA_Mid_out/1
  sfunction/236 -> [L466]
  [L467] -> TM_CCRGA_Req/1
  sfunction/237 -> [L467]
  [L468] -> term_TM_CCRGA_Req_MNMXDis/1
  sfunction/238 -> [L468]
  [L469] -> term_TM_CCRGA_Req_RefLo/1
  sfunction/239 -> [L469]
  [L470] -> term_TM_CCRTSHi_act/1
  sfunction/240 -> [L470]
  [L471] -> term_TM_CCRTSLo_act/1
  sfunction/241 -> [L471]
  [L472] -> term_TM_CCRTSMid_act/1
  sfunction/242 -> [L472]
  [L473] -> Ecm_CurCns48V/1
  sfunction/243 -> [L473]
  [L474] -> term_Epd_ClpmpMaxElPwr/1
  sfunction/244 -> [L474]
  [L475] -> term_Epd_EbstrMaxElPwr/1
  sfunction/245 -> [L475]
  [L476] -> term_Epd_PN48EcmMaxAllwdCur/1
  sfunction/246 -> [L476]
  [L477] -> term_Epd_PN48EcmSumElPwr/1
  sfunction/247 -> [L477]
  [L478] -> term_Epd_PwrMax48VRecupEzv/1
  sfunction/248 -> [L478]
  [L479] -> term_Net_Eboost_CurrLim/1
  sfunction/249 -> [L479]
  [L480] -> OilPump_Req_PWM/1
  sfunction/250 -> [L480]
  [L481] -> term_TmPcd_PwmOilPmpReq/1
  sfunction/251 -> [L481]
  [L482] -> ECU_RunOn_Mode_Req/1
  sfunction/252 -> [L482]
  [L483] -> term_Tm_EcuRunOnModReqRawFlg/1
  sfunction/253 -> [L483]
  [L484] -> term_TM_CCRGAEATHi/1
  sfunction/254 -> [L484]
  [L485] -> term_TM_CCRGAEATLo/1
  sfunction/255 -> [L485]
  [L486] -> term_TM_CCRGAEATMid/1
  sfunction/256 -> [L486]
  [L487] -> term_TM_CCRGA_Hi/1
  sfunction/257 -> [L487]
  [L488] -> term_TM_CCRGA_Lo/1
  sfunction/258 -> [L488]
  [L489] -> term_TM_CCRGA_Mid/1
  sfunction/259 -> [L489]
  [L490] -> term_TM_CCRGA_act/1
  sfunction/260 -> [L490]
  [L491] -> term_TM_ECT_Ref_Cntr_HT/1
  sfunction/261 -> [L491]
  [L492] -> term_TM_ECT_Ref_Cntr_LT/1
  sfunction/262 -> [L492]
  [L493] -> term_TOil_ShutOff/1
  sfunction/263 -> [L493]
  [L494] -> term_TmEcTpSp_CtrEcuTp0/1
  sfunction/264 -> [L494]
  [L495] -> term_TmEcTpSp_CtrEcuTp1/1
  sfunction/265 -> [L495]
  [L496] -> term_TmEcTpSp_CtrEcuTp2/1
  sfunction/266 -> [L496]
  [L497] -> term_TmEcTpSp_CtrEcuTp3/1
  sfunction/267 -> [L497]
  [L498] -> term_TmEcTpSp_CtrEcuTp4/1
  sfunction/268 -> [L498]
  [L499] -> term_TmEcTpSp_CtrEcuTp5/1
  sfunction/269 -> [L499]
  [L500] -> term_TmEcTpSp_CtrEcuTp6/1
  sfunction/270 -> [L500]
  [L501] -> term_TmEcTpSp_CtrEcuTp7/1
  sfunction/271 -> [L501]
  [L502] -> term_TmEcTpSp_CtrEcuTp8/1
  sfunction/272 -> [L502]
  [L503] -> term_TmEcTpSp_CtrEcuTp9/1
  sfunction/273 -> [L503]
  [L504] -> term_TmEcTpSp_TpEcuCtrDiRam/1
  sfunction/274 -> [L504]
  [L505] -> term_TmHi_FacTCor2Ee/1
  sfunction/275 -> [L505]
  [L506] -> term_TmPcdLrng_CtlrFctCoefY100/1
  sfunction/276 -> [L506]
  [L507] -> term_TmPcdLrng_CtlrFctCoefY20/1
  sfunction/277 -> [L507]
  [L508] -> term_TmPcd_EepromPDeacvnOdoS/1
  sfunction/278 -> [L508]
  [L509] -> term_TmPmp_TpQhtTchDram/1
  sfunction/279 -> [L509]
  [L510] -> term_ut_Trigger_Cyl_Cntr/1
  sfunction/280 -> [L510]
  [L329] -> term_EngSys_PGasIntkAry/1
  [L332] -> term_EngSys_QInjAry/1
  [L335] -> term_EngSys_TpEngAry/1
  [L338] -> term_EngSys_TpEngStrtAry/1
  [L341] -> term_EngSys_TpGasIntkAry/1
  ECTOut/1 -> Dlay_ECTOut/1
  EngShutOff_Time/1 -> Dlay_EngShutOff_Time/1
  Exh_Temp/1 -> Dlay_Exh_Temp/1
  FirstStrt_Mode_EE/1 -> Dlay_FirstStrt_Mode_EE/1
  IgnSwRun_Mode/1 -> Dlay_IgnSwRun_Mode/1
  LIN_CF_Spd_Req/1 -> Dlay_LIN_CF_Spd_Req/1
  Shuttr_Pos_Req_I/1 -> Dlay_Shuttr_Pos_Req_I/1
  TM_ShttrDeIcing_ECTRef_I/1 -> Dlay_TM_ShttrDeIcing_ECTRef_I/1
  TM_Shttr_TjaErrIrrv_LIN/1 -> Dlay_TM_Shttr_TjaErrIrrv_LIN/1
  TmClpmp_LtCcrGbRsgTpQvolReq/1 -> Dlay_TmClpmp_LtCcrGbRsgTpQvolReq/1
  TmFan_MalfFlg/1 -> Dlay_TmFan_MalfFlg/1
  TmHiTp_ThOpenSts/1 -> Dlay_TmHiTp_ThOpenSts/1
  Tm_FlgEngOilHiPReq/1 -> Dlay_Tm_FlgEngOilHiPReq/1
  flg_ChrgrAirCcrAcv/1 -> Dlay_flg_ChrgrAirCcrAcv/1
  flg_PAFGCoolFanLinMod/1 -> Dlay_flg_PAFGCoolFanLinMod/1
  perc_PAFGCoolFanLinReq/1 -> Dlay_perc_PAFGCoolFanLinReq/1
